simulink model "x00_AeroDynamicModelMainAssembly"  (R2016a)
settings: Solver=ode23t  StartTime=0.0  StopTime=10.0  MaxStep=0.1  RelTol=1e-3
model workspace: external: MATLAB File C:\Users\szhang\2016 ACT- Quanser\Aero Dynamic Model Export\x00_AeroDynamicModelMainAssembly_DataFile1.m (data not in the file)
undefined symbols (not defined in the file or in its folder): _AICAD8418WBRMZ_Default_sldprt, _AICBCR421UW67_Default_sldprt, _C0402100n25V_Default_sldprt, _C040210n25V_Default_sldprt, _C040212p50VC0G_Default_sldprt, _C06031u35V_Default_sldprt, _C06032u216V_Default_sldprt, _C100U50VEEEFC1H101P_Default_sldprt, _C12064u750V_01_sldprt, _C121010U50V_Default_sldprt, _COMMCYUSB2014BZXC_Default_sldprt, _COMMON_01_sldprt, _COMMON_Default_sldprt, _CONNFUSBBSMT_01_sldprt, _CONNMDF3A12P2DSA_Default_sldprt, _CONNMDF3A4P2DSA_Default_sldprt, _CONNMDF3A6P2DS_Default_sldprt, _CONNMDF3A9P2DS_Default_sldprt, _CONNMODULAR8P8CTOP_Default_sldprt, _CONNPJ102BH_Default_sldprt, _CP6100U50VC0G_Default_sldprt, _CPLD5M80ZE64C5_Default_sldprt, _DB560C13F_01_sldprt, _Default_sldprt, _DSMBJ5361BTP_Default_sldprt, _EEPROMAT24CM01_Default_sldprt, _FBBLM21PG221SN1D_01_sldprt, _FBMPZ2012S601A_01_sldprt, _LED3mmRedGreenRA_Default_sldprt, _LEDLTRBGFSFRedGreenBlue_Default_sldprt, _LOGICNCP361SNT1G_Default_sldprt, _LOGICNOTSN74LVC3G14DCU_Default_sldprt, _OPL6206QTR_Default_sldprt, _OSC40000MHZ_Default_sldprt, _R0402100K_Default_sldprt, _R040210K0_Default_sldprt, _R04021K00_Default_sldprt, _R0402200R_Default_sldprt, _R040222R0_Default_sldprt, _R04026K04_Default_sldprt, _R0402DNP_Default_sldprt, _RA40R0_Default_sldprt, _RA41K005, _TP16258543_01_sldprt, _TVSUNI28V_Default_sldprt, _TVSUNI53V_Default_sldprt, _VREGAP733333SAG7_Default_sldprt, _VREGLTM8022EVPBF_Default_sldprt, _VREGPAM3112DAB120_Default_sldprt, _VREGTPS79318DBVR_01_sldprt, _XTAL192MHZNX2520SA_Default_sldprt, BGA121, CAP, CEEEFC1H101P, CONNFUSBBSMT, CONNMDF3A12P2DSA, CONNMDF3A4P2DSA, CONNMDF3A6P2DS, CONNMDF3A9P2DS, CONNModular8P8C ... (+31)
libraries: sm_lib x1879, nesl_utility x1
(part 29 of 35)

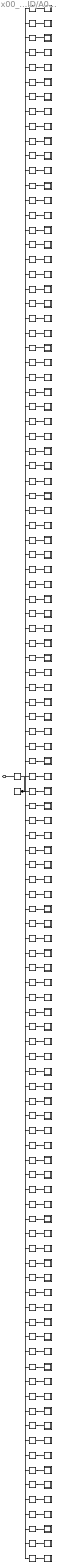
== system x00_AeroDynamicModelMainAssembly/x03_Aero_Dynamic_Model_Pivot_1_RIGID/A002_759_1_RIGID/A002_758_1_RIGID/C006_285_1_RIGID ==
  C006_285_1_RIGID : Subsystem
  CEEEFC1H101P_C100U50VEEEFC1H101P_1_RIGID : Subsystem
  CONNMDF3A6P2DS_CONNMDF3A6P2DS_1_RIGID : Subsystem
  CONNMDF3A6P2DS_CONNMDF3A6P2DS_2_RIGID : Subsystem
  CONNMDF3A9P2DS_CONNMDF3A9P2DS_1_RIGID : Subsystem
  DDO214AA_DSMBJ5361BTP_1_RIGID : Subsystem
  DDO214AB_DB560C13F_1_RIGID : Subsystem
  LGA16_3x3x086mm_ACCGYROLSM6DS0_1_RIGID : Subsystem
  MSOP10_COMMON_1_RIGID : Subsystem
  MSOP8Q_AICAD8418WBRMZ_1_RIGID : Subsystem
  MSOP8Q_AICAD8418WBRMZ_2_RIGID : Subsystem
  MSOP8Q_AICAD8418WBRMZ_3_RIGID : Subsystem
  MSOP8Q_AICAD8418WBRMZ_4_RIGID : Subsystem
  OSCECS20xx_OSC40000MHZ_1_RIGID : Subsystem
  RARRAYYC124_RA40R0_1_RIGID : Subsystem
  RARRAYYC124_RA40R0_2_RIGID : Subsystem
  RARRAYYC124_RA40R0_3_RIGID : Subsystem
  RARRAYYC124_RA40R0_4_RIGID : Subsystem
  RARRAYYC124_RA41K005_1_RIGID : Subsystem
  RARRAYYC124_RA41K005_2_RIGID : Subsystem
  ReferenceFrame : sm_lib/Frames and Transforms/Reference Frame
  SOT235_COMMON_1_RIGID : Subsystem
  SOT235_COMMON_2_RIGID : Subsystem
  SOT23_COMMON_1_RIGID : Subsystem
  SOT23_COMMON_2_RIGID : Subsystem
  SOT23_COMMON_3_RIGID : Subsystem
  TP16258543_TP16258543_1_RIGID : Subsystem
  TP16258543_TP16258543_2_RIGID : Subsystem
  TP16258543_TP16258543_3_RIGID : Subsystem
  TP16258543_TP16258543_4_RIGID : Subsystem
  TP16258543_TP16258543_5_RIGID : Subsystem
  TP16258543_TP16258543_6_RIGID : Subsystem
  TQFP144Max_V_CPLD_ground_pins_CPLD5M1270ZT144C5N_1_RIGID : Subsystem
  Transform : sm_lib/Frames and Transforms/Rigid Transform  TranslationMethod=Cartesian  TranslationLengthUnit=in  TranslationStandardAxis=+Z  TranslationStandardOffset=0  TranslationCartesianOffset=smiData.RigidTransform(427).translation  TranslationROffset=0  TranslationROffsetUnits=m  TranslationZOffset=0  TranslationZOffsetUnits=m  TranslationThetaOffset=0  TranslationThetaOffsetUnits=deg  RotationMethod=ArbitraryAxis  RotationAngleUnits=rad  RotationStandardAxis=+Z  RotationAngle=smiData.RigidTransform(427).angle  RotationArbitraryAxis=smiData.RigidTransform(427).axis  FollAlignAxisA=+X  BaseAlignAxisA=+Y  FollAlignAxisB=+Y  BaseAlignAxisB=+Z  RotationSequenceAxes=FollowerAxes  RotationSequence=XYX  RotationSequenceAngles=[0 0 0]  RotationSequenceAnglesUnits=deg  RotationMatrix=[1 0 0; 0 1 0; 0 0 1]
  Transform1 : sm_lib/Frames and Transforms/Rigid Transform  TranslationMethod=Cartesian  TranslationLengthUnit=in  TranslationStandardAxis=+Z  TranslationStandardOffset=0  TranslationCartesianOffset=smiData.RigidTransform(428).translation  TranslationROffset=0  TranslationROffsetUnits=m  TranslationZOffset=0  TranslationZOffsetUnits=m  TranslationThetaOffset=0  TranslationThetaOffsetUnits=deg  RotationMethod=ArbitraryAxis  RotationAngleUnits=rad  RotationStandardAxis=+Z  RotationAngle=smiData.RigidTransform(428).angle  RotationArbitraryAxis=smiData.RigidTransform(428).axis  FollAlignAxisA=+X  BaseAlignAxisA=+Y  FollAlignAxisB=+Y  BaseAlignAxisB=+Z  RotationSequenceAxes=FollowerAxes  RotationSequence=XYX  RotationSequenceAngles=[0 0 0]  RotationSequenceAnglesUnits=deg  RotationMatrix=[1 0 0; 0 1 0; 0 0 1]
  Transform10 : sm_lib/Frames and Transforms/Rigid Transform  TranslationMethod=Cartesian  TranslationLengthUnit=in  TranslationStandardAxis=+Z  TranslationStandardOffset=0  TranslationCartesianOffset=smiData.RigidTransform(437).translation  TranslationROffset=0  TranslationROffsetUnits=m  TranslationZOffset=0  TranslationZOffsetUnits=m  TranslationThetaOffset=0  TranslationThetaOffsetUnits=deg  RotationMethod=ArbitraryAxis  RotationAngleUnits=rad  RotationStandardAxis=+Z  RotationAngle=smiData.RigidTransform(437).angle  RotationArbitraryAxis=smiData.RigidTransform(437).axis  FollAlignAxisA=+X  BaseAlignAxisA=+Y  FollAlignAxisB=+Y  BaseAlignAxisB=+Z  RotationSequenceAxes=FollowerAxes  RotationSequence=XYX  RotationSequenceAngles=[0 0 0]  RotationSequenceAnglesUnits=deg  RotationMatrix=[1 0 0; 0 1 0; 0 0 1]
  Transform100 : sm_lib/Frames and Transforms/Rigid Transform  TranslationMethod=Cartesian  TranslationLengthUnit=in  TranslationStandardAxis=+Z  TranslationStandardOffset=0  TranslationCartesianOffset=smiData.RigidTransform(527).translation  TranslationROffset=0  TranslationROffsetUnits=m  TranslationZOffset=0  TranslationZOffsetUnits=m  TranslationThetaOffset=0  TranslationThetaOffsetUnits=deg  RotationMethod=ArbitraryAxis  RotationAngleUnits=rad  RotationStandardAxis=+Z  RotationAngle=smiData.RigidTransform(527).angle  RotationArbitraryAxis=smiData.RigidTransform(527).axis  FollAlignAxisA=+X  BaseAlignAxisA=+Y  FollAlignAxisB=+Y  BaseAlignAxisB=+Z  RotationSequenceAxes=FollowerAxes  RotationSequence=XYX  RotationSequenceAngles=[0 0 0]  RotationSequenceAnglesUnits=deg  RotationMatrix=[1 0 0; 0 1 0; 0 0 1]
  Transform101 : sm_lib/Frames and Transforms/Rigid Transform  TranslationMethod=Cartesian  TranslationLengthUnit=in  TranslationStandardAxis=+Z  TranslationStandardOffset=0  TranslationCartesianOffset=smiData.RigidTransform(528).translation  TranslationROffset=0  TranslationROffsetUnits=m  TranslationZOffset=0  TranslationZOffsetUnits=m  TranslationThetaOffset=0  TranslationThetaOffsetUnits=deg  RotationMethod=ArbitraryAxis  RotationAngleUnits=rad  RotationStandardAxis=+Z  RotationAngle=smiData.RigidTransform(528).angle  RotationArbitraryAxis=smiData.RigidTransform(528).axis  FollAlignAxisA=+X  BaseAlignAxisA=+Y  FollAlignAxisB=+Y  BaseAlignAxisB=+Z  RotationSequenceAxes=FollowerAxes  RotationSequence=XYX  RotationSequenceAngles=[0 0 0]  RotationSequenceAnglesUnits=deg  RotationMatrix=[1 0 0; 0 1 0; 0 0 1]
  Transform102 : sm_lib/Frames and Transforms/Rigid Transform  TranslationMethod=Cartesian  TranslationLengthUnit=in  TranslationStandardAxis=+Z  TranslationStandardOffset=0  TranslationCartesianOffset=smiData.RigidTransform(529).translation  TranslationROffset=0  TranslationROffsetUnits=m  TranslationZOffset=0  TranslationZOffsetUnits=m  TranslationThetaOffset=0  TranslationThetaOffsetUnits=deg  RotationMethod=ArbitraryAxis  RotationAngleUnits=rad  RotationStandardAxis=+Z  RotationAngle=smiData.RigidTransform(529).angle  RotationArbitraryAxis=smiData.RigidTransform(529).axis  FollAlignAxisA=+X  BaseAlignAxisA=+Y  FollAlignAxisB=+Y  BaseAlignAxisB=+Z  RotationSequenceAxes=FollowerAxes  RotationSequence=XYX  RotationSequenceAngles=[0 0 0]  RotationSequenceAnglesUnits=deg  RotationMatrix=[1 0 0; 0 1 0; 0 0 1]
  Transform103 : sm_lib/Frames and Transforms/Rigid Transform  TranslationMethod=Cartesian  TranslationLengthUnit=in  TranslationStandardAxis=+Z  TranslationStandardOffset=0  TranslationCartesianOffset=smiData.RigidTransform(530).translation  TranslationROffset=0  TranslationROffsetUnits=m  TranslationZOffset=0  TranslationZOffsetUnits=m  TranslationThetaOffset=0  TranslationThetaOffsetUnits=deg  RotationMethod=ArbitraryAxis  RotationAngleUnits=rad  RotationStandardAxis=+Z  RotationAngle=smiData.RigidTransform(530).angle  RotationArbitraryAxis=smiData.RigidTransform(530).axis  FollAlignAxisA=+X  BaseAlignAxisA=+Y  FollAlignAxisB=+Y  BaseAlignAxisB=+Z  RotationSequenceAxes=FollowerAxes  RotationSequence=XYX  RotationSequenceAngles=[0 0 0]  RotationSequenceAnglesUnits=deg  RotationMatrix=[1 0 0; 0 1 0; 0 0 1]
  Transform104 : sm_lib/Frames and Transforms/Rigid Transform  TranslationMethod=Cartesian  TranslationLengthUnit=in  TranslationStandardAxis=+Z  TranslationStandardOffset=0  TranslationCartesianOffset=smiData.RigidTransform(531).translation  TranslationROffset=0  TranslationROffsetUnits=m  TranslationZOffset=0  TranslationZOffsetUnits=m  TranslationThetaOffset=0  TranslationThetaOffsetUnits=deg  RotationMethod=ArbitraryAxis  RotationAngleUnits=rad  RotationStandardAxis=+Z  RotationAngle=smiData.RigidTransform(531).angle  RotationArbitraryAxis=smiData.RigidTransform(531).axis  FollAlignAxisA=+X  BaseAlignAxisA=+Y  FollAlignAxisB=+Y  BaseAlignAxisB=+Z  RotationSequenceAxes=FollowerAxes  RotationSequence=XYX  RotationSequenceAngles=[0 0 0]  RotationSequenceAnglesUnits=deg  RotationMatrix=[1 0 0; 0 1 0; 0 0 1]
  Transform105 : sm_lib/Frames and Transforms/Rigid Transform  TranslationMethod=Cartesian  TranslationLengthUnit=in  TranslationStandardAxis=+Z  TranslationStandardOffset=0  TranslationCartesianOffset=smiData.RigidTransform(532).translation  TranslationROffset=0  TranslationROffsetUnits=m  TranslationZOffset=0  TranslationZOffsetUnits=m  TranslationThetaOffset=0  TranslationThetaOffsetUnits=deg  RotationMethod=ArbitraryAxis  RotationAngleUnits=rad  RotationStandardAxis=+Z  RotationAngle=smiData.RigidTransform(532).angle  RotationArbitraryAxis=smiData.RigidTransform(532).axis  FollAlignAxisA=+X  BaseAlignAxisA=+Y  FollAlignAxisB=+Y  BaseAlignAxisB=+Z  RotationSequenceAxes=FollowerAxes  RotationSequence=XYX  RotationSequenceAngles=[0 0 0]  RotationSequenceAnglesUnits=deg  RotationMatrix=[1 0 0; 0 1 0; 0 0 1]
  Transform106 : sm_lib/Frames and Transforms/Rigid Transform  TranslationMethod=Cartesian  TranslationLengthUnit=in  TranslationStandardAxis=+Z  TranslationStandardOffset=0  TranslationCartesianOffset=smiData.RigidTransform(533).translation  TranslationROffset=0  TranslationROffsetUnits=m  TranslationZOffset=0  TranslationZOffsetUnits=m  TranslationThetaOffset=0  TranslationThetaOffsetUnits=deg  RotationMethod=ArbitraryAxis  RotationAngleUnits=rad  RotationStandardAxis=+Z  RotationAngle=smiData.RigidTransform(533).angle  RotationArbitraryAxis=smiData.RigidTransform(533).axis  FollAlignAxisA=+X  BaseAlignAxisA=+Y  FollAlignAxisB=+Y  BaseAlignAxisB=+Z  RotationSequenceAxes=FollowerAxes  RotationSequence=XYX  RotationSequenceAngles=[0 0 0]  RotationSequenceAnglesUnits=deg  RotationMatrix=[1 0 0; 0 1 0; 0 0 1]
  Transform11 : sm_lib/Frames and Transforms/Rigid Transform  TranslationMethod=Cartesian  TranslationLengthUnit=in  TranslationStandardAxis=+Z  TranslationStandardOffset=0  TranslationCartesianOffset=smiData.RigidTransform(438).translation  TranslationROffset=0  TranslationROffsetUnits=m  TranslationZOffset=0  TranslationZOffsetUnits=m  TranslationThetaOffset=0  TranslationThetaOffsetUnits=deg  RotationMethod=ArbitraryAxis  RotationAngleUnits=rad  RotationStandardAxis=+Z  RotationAngle=smiData.RigidTransform(438).angle  RotationArbitraryAxis=smiData.RigidTransform(438).axis  FollAlignAxisA=+X  BaseAlignAxisA=+Y  FollAlignAxisB=+Y  BaseAlignAxisB=+Z  RotationSequenceAxes=FollowerAxes  RotationSequence=XYX  RotationSequenceAngles=[0 0 0]  RotationSequenceAnglesUnits=deg  RotationMatrix=[1 0 0; 0 1 0; 0 0 1]
  Transform12 : sm_lib/Frames and Transforms/Rigid Transform  TranslationMethod=Cartesian  TranslationLengthUnit=in  TranslationStandardAxis=+Z  TranslationStandardOffset=0  TranslationCartesianOffset=smiData.RigidTransform(439).translation  TranslationROffset=0  TranslationROffsetUnits=m  TranslationZOffset=0  TranslationZOffsetUnits=m  TranslationThetaOffset=0  TranslationThetaOffsetUnits=deg  RotationMethod=ArbitraryAxis  RotationAngleUnits=rad  RotationStandardAxis=+Z  RotationAngle=smiData.RigidTransform(439).angle  RotationArbitraryAxis=smiData.RigidTransform(439).axis  FollAlignAxisA=+X  BaseAlignAxisA=+Y  FollAlignAxisB=+Y  BaseAlignAxisB=+Z  RotationSequenceAxes=FollowerAxes  RotationSequence=XYX  RotationSequenceAngles=[0 0 0]  RotationSequenceAnglesUnits=deg  RotationMatrix=[1 0 0; 0 1 0; 0 0 1]
  Transform13 : sm_lib/Frames and Transforms/Rigid Transform  TranslationMethod=Cartesian  TranslationLengthUnit=in  TranslationStandardAxis=+Z  TranslationStandardOffset=0  TranslationCartesianOffset=smiData.RigidTransform(440).translation  TranslationROffset=0  TranslationROffsetUnits=m  TranslationZOffset=0  TranslationZOffsetUnits=m  TranslationThetaOffset=0  TranslationThetaOffsetUnits=deg  RotationMethod=ArbitraryAxis  RotationAngleUnits=rad  RotationStandardAxis=+Z  RotationAngle=smiData.RigidTransform(440).angle  RotationArbitraryAxis=smiData.RigidTransform(440).axis  FollAlignAxisA=+X  BaseAlignAxisA=+Y  FollAlignAxisB=+Y  BaseAlignAxisB=+Z  RotationSequenceAxes=FollowerAxes  RotationSequence=XYX  RotationSequenceAngles=[0 0 0]  RotationSequenceAnglesUnits=deg  RotationMatrix=[1 0 0; 0 1 0; 0 0 1]
  Transform14 : sm_lib/Frames and Transforms/Rigid Transform  TranslationMethod=Cartesian  TranslationLengthUnit=in  TranslationStandardAxis=+Z  TranslationStandardOffset=0  TranslationCartesianOffset=smiData.RigidTransform(441).translation  TranslationROffset=0  TranslationROffsetUnits=m  TranslationZOffset=0  TranslationZOffsetUnits=m  TranslationThetaOffset=0  TranslationThetaOffsetUnits=deg  RotationMethod=ArbitraryAxis  RotationAngleUnits=rad  RotationStandardAxis=+Z  RotationAngle=smiData.RigidTransform(441).angle  RotationArbitraryAxis=smiData.RigidTransform(441).axis  FollAlignAxisA=+X  BaseAlignAxisA=+Y  FollAlignAxisB=+Y  BaseAlignAxisB=+Z  RotationSequenceAxes=FollowerAxes  RotationSequence=XYX  RotationSequenceAngles=[0 0 0]  RotationSequenceAnglesUnits=deg  RotationMatrix=[1 0 0; 0 1 0; 0 0 1]
  Transform15 : sm_lib/Frames and Transforms/Rigid Transform  TranslationMethod=Cartesian  TranslationLengthUnit=in  TranslationStandardAxis=+Z  TranslationStandardOffset=0  TranslationCartesianOffset=smiData.RigidTransform(442).translation  TranslationROffset=0  TranslationROffsetUnits=m  TranslationZOffset=0  TranslationZOffsetUnits=m  TranslationThetaOffset=0  TranslationThetaOffsetUnits=deg  RotationMethod=ArbitraryAxis  RotationAngleUnits=rad  RotationStandardAxis=+Z  RotationAngle=smiData.RigidTransform(442).angle  RotationArbitraryAxis=smiData.RigidTransform(442).axis  FollAlignAxisA=+X  BaseAlignAxisA=+Y  FollAlignAxisB=+Y  BaseAlignAxisB=+Z  RotationSequenceAxes=FollowerAxes  RotationSequence=XYX  RotationSequenceAngles=[0 0 0]  RotationSequenceAnglesUnits=deg  RotationMatrix=[1 0 0; 0 1 0; 0 0 1]
  Transform16 : sm_lib/Frames and Transforms/Rigid Transform  TranslationMethod=Cartesian  TranslationLengthUnit=in  TranslationStandardAxis=+Z  TranslationStandardOffset=0  TranslationCartesianOffset=smiData.RigidTransform(443).translation  TranslationROffset=0  TranslationROffsetUnits=m  TranslationZOffset=0  TranslationZOffsetUnits=m  TranslationThetaOffset=0  TranslationThetaOffsetUnits=deg  RotationMethod=ArbitraryAxis  RotationAngleUnits=rad  RotationStandardAxis=+Z  RotationAngle=smiData.RigidTransform(443).angle  RotationArbitraryAxis=smiData.RigidTransform(443).axis  FollAlignAxisA=+X  BaseAlignAxisA=+Y  FollAlignAxisB=+Y  BaseAlignAxisB=+Z  RotationSequenceAxes=FollowerAxes  RotationSequence=XYX  RotationSequenceAngles=[0 0 0]  RotationSequenceAnglesUnits=deg  RotationMatrix=[1 0 0; 0 1 0; 0 0 1]
  Transform17 : sm_lib/Frames and Transforms/Rigid Transform  TranslationMethod=Cartesian  TranslationLengthUnit=in  TranslationStandardAxis=+Z  TranslationStandardOffset=0  TranslationCartesianOffset=smiData.RigidTransform(444).translation  TranslationROffset=0  TranslationROffsetUnits=m  TranslationZOffset=0  TranslationZOffsetUnits=m  TranslationThetaOffset=0  TranslationThetaOffsetUnits=deg  RotationMethod=ArbitraryAxis  RotationAngleUnits=rad  RotationStandardAxis=+Z  RotationAngle=smiData.RigidTransform(444).angle  RotationArbitraryAxis=smiData.RigidTransform(444).axis  FollAlignAxisA=+X  BaseAlignAxisA=+Y  FollAlignAxisB=+Y  BaseAlignAxisB=+Z  RotationSequenceAxes=FollowerAxes  RotationSequence=XYX  RotationSequenceAngles=[0 0 0]  RotationSequenceAnglesUnits=deg  RotationMatrix=[1 0 0; 0 1 0; 0 0 1]
  Transform18 : sm_lib/Frames and Transforms/Rigid Transform  TranslationMethod=Cartesian  TranslationLengthUnit=in  TranslationStandardAxis=+Z  TranslationStandardOffset=0  TranslationCartesianOffset=smiData.RigidTransform(445).translation  TranslationROffset=0  TranslationROffsetUnits=m  TranslationZOffset=0  TranslationZOffsetUnits=m  TranslationThetaOffset=0  TranslationThetaOffsetUnits=deg  RotationMethod=ArbitraryAxis  RotationAngleUnits=rad  RotationStandardAxis=+Z  RotationAngle=smiData.RigidTransform(445).angle  RotationArbitraryAxis=smiData.RigidTransform(445).axis  FollAlignAxisA=+X  BaseAlignAxisA=+Y  FollAlignAxisB=+Y  BaseAlignAxisB=+Z  RotationSequenceAxes=FollowerAxes  RotationSequence=XYX  RotationSequenceAngles=[0 0 0]  RotationSequenceAnglesUnits=deg  RotationMatrix=[1 0 0; 0 1 0; 0 0 1]
  Transform19 : sm_lib/Frames and Transforms/Rigid Transform  TranslationMethod=Cartesian  TranslationLengthUnit=in  TranslationStandardAxis=+Z  TranslationStandardOffset=0  TranslationCartesianOffset=smiData.RigidTransform(446).translation  TranslationROffset=0  TranslationROffsetUnits=m  TranslationZOffset=0  TranslationZOffsetUnits=m  TranslationThetaOffset=0  TranslationThetaOffsetUnits=deg  RotationMethod=ArbitraryAxis  RotationAngleUnits=rad  RotationStandardAxis=+Z  RotationAngle=smiData.RigidTransform(446).angle  RotationArbitraryAxis=smiData.RigidTransform(446).axis  FollAlignAxisA=+X  BaseAlignAxisA=+Y  FollAlignAxisB=+Y  BaseAlignAxisB=+Z  RotationSequenceAxes=FollowerAxes  RotationSequence=XYX  RotationSequenceAngles=[0 0 0]  RotationSequenceAnglesUnits=deg  RotationMatrix=[1 0 0; 0 1 0; 0 0 1]
  Transform2 : sm_lib/Frames and Transforms/Rigid Transform  TranslationMethod=Cartesian  TranslationLengthUnit=in  TranslationStandardAxis=+Z  TranslationStandardOffset=0  TranslationCartesianOffset=smiData.RigidTransform(429).translation  TranslationROffset=0  TranslationROffsetUnits=m  TranslationZOffset=0  TranslationZOffsetUnits=m  TranslationThetaOffset=0  TranslationThetaOffsetUnits=deg  RotationMethod=ArbitraryAxis  RotationAngleUnits=rad  RotationStandardAxis=+Z  RotationAngle=smiData.RigidTransform(429).angle  RotationArbitraryAxis=smiData.RigidTransform(429).axis  FollAlignAxisA=+X  BaseAlignAxisA=+Y  FollAlignAxisB=+Y  BaseAlignAxisB=+Z  RotationSequenceAxes=FollowerAxes  RotationSequence=XYX  RotationSequenceAngles=[0 0 0]  RotationSequenceAnglesUnits=deg  RotationMatrix=[1 0 0; 0 1 0; 0 0 1]
  Transform20 : sm_lib/Frames and Transforms/Rigid Transform  TranslationMethod=Cartesian  TranslationLengthUnit=in  TranslationStandardAxis=+Z  TranslationStandardOffset=0  TranslationCartesianOffset=smiData.RigidTransform(447).translation  TranslationROffset=0  TranslationROffsetUnits=m  TranslationZOffset=0  TranslationZOffsetUnits=m  TranslationThetaOffset=0  TranslationThetaOffsetUnits=deg  RotationMethod=ArbitraryAxis  RotationAngleUnits=rad  RotationStandardAxis=+Z  RotationAngle=smiData.RigidTransform(447).angle  RotationArbitraryAxis=smiData.RigidTransform(447).axis  FollAlignAxisA=+X  BaseAlignAxisA=+Y  FollAlignAxisB=+Y  BaseAlignAxisB=+Z  RotationSequenceAxes=FollowerAxes  RotationSequence=XYX  RotationSequenceAngles=[0 0 0]  RotationSequenceAnglesUnits=deg  RotationMatrix=[1 0 0; 0 1 0; 0 0 1]
  Transform21 : sm_lib/Frames and Transforms/Rigid Transform  TranslationMethod=Cartesian  TranslationLengthUnit=in  TranslationStandardAxis=+Z  TranslationStandardOffset=0  TranslationCartesianOffset=smiData.RigidTransform(448).translation  TranslationROffset=0  TranslationROffsetUnits=m  TranslationZOffset=0  TranslationZOffsetUnits=m  TranslationThetaOffset=0  TranslationThetaOffsetUnits=deg  RotationMethod=ArbitraryAxis  RotationAngleUnits=rad  RotationStandardAxis=+Z  RotationAngle=smiData.RigidTransform(448).angle  RotationArbitraryAxis=smiData.RigidTransform(448).axis  FollAlignAxisA=+X  BaseAlignAxisA=+Y  FollAlignAxisB=+Y  BaseAlignAxisB=+Z  RotationSequenceAxes=FollowerAxes  RotationSequence=XYX  RotationSequenceAngles=[0 0 0]  RotationSequenceAnglesUnits=deg  RotationMatrix=[1 0 0; 0 1 0; 0 0 1]
  Transform22 : sm_lib/Frames and Transforms/Rigid Transform  TranslationMethod=Cartesian  TranslationLengthUnit=in  TranslationStandardAxis=+Z  TranslationStandardOffset=0  TranslationCartesianOffset=smiData.RigidTransform(449).translation  TranslationROffset=0  TranslationROffsetUnits=m  TranslationZOffset=0  TranslationZOffsetUnits=m  TranslationThetaOffset=0  TranslationThetaOffsetUnits=deg  RotationMethod=ArbitraryAxis  RotationAngleUnits=rad  RotationStandardAxis=+Z  RotationAngle=smiData.RigidTransform(449).angle  RotationArbitraryAxis=smiData.RigidTransform(449).axis  FollAlignAxisA=+X  BaseAlignAxisA=+Y  FollAlignAxisB=+Y  BaseAlignAxisB=+Z  RotationSequenceAxes=FollowerAxes  RotationSequence=XYX  RotationSequenceAngles=[0 0 0]  RotationSequenceAnglesUnits=deg  RotationMatrix=[1 0 0; 0 1 0; 0 0 1]
  Transform23 : sm_lib/Frames and Transforms/Rigid Transform  TranslationMethod=Cartesian  TranslationLengthUnit=in  TranslationStandardAxis=+Z  TranslationStandardOffset=0  TranslationCartesianOffset=smiData.RigidTransform(450).translation  TranslationROffset=0  TranslationROffsetUnits=m  TranslationZOffset=0  TranslationZOffsetUnits=m  TranslationThetaOffset=0  TranslationThetaOffsetUnits=deg  RotationMethod=ArbitraryAxis  RotationAngleUnits=rad  RotationStandardAxis=+Z  RotationAngle=smiData.RigidTransform(450).angle  RotationArbitraryAxis=smiData.RigidTransform(450).axis  FollAlignAxisA=+X  BaseAlignAxisA=+Y  FollAlignAxisB=+Y  BaseAlignAxisB=+Z  RotationSequenceAxes=FollowerAxes  RotationSequence=XYX  RotationSequenceAngles=[0 0 0]  RotationSequenceAnglesUnits=deg  RotationMatrix=[1 0 0; 0 1 0; 0 0 1]
  Transform24 : sm_lib/Frames and Transforms/Rigid Transform  TranslationMethod=Cartesian  TranslationLengthUnit=in  TranslationStandardAxis=+Z  TranslationStandardOffset=0  TranslationCartesianOffset=smiData.RigidTransform(451).translation  TranslationROffset=0  TranslationROffsetUnits=m  TranslationZOffset=0  TranslationZOffsetUnits=m  TranslationThetaOffset=0  TranslationThetaOffsetUnits=deg  RotationMethod=ArbitraryAxis  RotationAngleUnits=rad  RotationStandardAxis=+Z  RotationAngle=smiData.RigidTransform(451).angle  RotationArbitraryAxis=smiData.RigidTransform(451).axis  FollAlignAxisA=+X  BaseAlignAxisA=+Y  FollAlignAxisB=+Y  BaseAlignAxisB=+Z  RotationSequenceAxes=FollowerAxes  RotationSequence=XYX  RotationSequenceAngles=[0 0 0]  RotationSequenceAnglesUnits=deg  RotationMatrix=[1 0 0; 0 1 0; 0 0 1]
  Transform25 : sm_lib/Frames and Transforms/Rigid Transform  TranslationMethod=Cartesian  TranslationLengthUnit=in  TranslationStandardAxis=+Z  TranslationStandardOffset=0  TranslationCartesianOffset=smiData.RigidTransform(452).translation  TranslationROffset=0  TranslationROffsetUnits=m  TranslationZOffset=0  TranslationZOffsetUnits=m  TranslationThetaOffset=0  TranslationThetaOffsetUnits=deg  RotationMethod=ArbitraryAxis  RotationAngleUnits=rad  RotationStandardAxis=+Z  RotationAngle=smiData.RigidTransform(452).angle  RotationArbitraryAxis=smiData.RigidTransform(452).axis  FollAlignAxisA=+X  BaseAlignAxisA=+Y  FollAlignAxisB=+Y  BaseAlignAxisB=+Z  RotationSequenceAxes=FollowerAxes  RotationSequence=XYX  RotationSequenceAngles=[0 0 0]  RotationSequenceAnglesUnits=deg  RotationMatrix=[1 0 0; 0 1 0; 0 0 1]
  Transform26 : sm_lib/Frames and Transforms/Rigid Transform  TranslationMethod=Cartesian  TranslationLengthUnit=in  TranslationStandardAxis=+Z  TranslationStandardOffset=0  TranslationCartesianOffset=smiData.RigidTransform(453).translation  TranslationROffset=0  TranslationROffsetUnits=m  TranslationZOffset=0  TranslationZOffsetUnits=m  TranslationThetaOffset=0  TranslationThetaOffsetUnits=deg  RotationMethod=ArbitraryAxis  RotationAngleUnits=rad  RotationStandardAxis=+Z  RotationAngle=smiData.RigidTransform(453).angle  RotationArbitraryAxis=smiData.RigidTransform(453).axis  FollAlignAxisA=+X  BaseAlignAxisA=+Y  FollAlignAxisB=+Y  BaseAlignAxisB=+Z  RotationSequenceAxes=FollowerAxes  RotationSequence=XYX  RotationSequenceAngles=[0 0 0]  RotationSequenceAnglesUnits=deg  RotationMatrix=[1 0 0; 0 1 0; 0 0 1]
  Transform27 : sm_lib/Frames and Transforms/Rigid Transform  TranslationMethod=Cartesian  TranslationLengthUnit=in  TranslationStandardAxis=+Z  TranslationStandardOffset=0  TranslationCartesianOffset=smiData.RigidTransform(454).translation  TranslationROffset=0  TranslationROffsetUnits=m  TranslationZOffset=0  TranslationZOffsetUnits=m  TranslationThetaOffset=0  TranslationThetaOffsetUnits=deg  RotationMethod=ArbitraryAxis  RotationAngleUnits=rad  RotationStandardAxis=+Z  RotationAngle=smiData.RigidTransform(454).angle  RotationArbitraryAxis=smiData.RigidTransform(454).axis  FollAlignAxisA=+X  BaseAlignAxisA=+Y  FollAlignAxisB=+Y  BaseAlignAxisB=+Z  RotationSequenceAxes=FollowerAxes  RotationSequence=XYX  RotationSequenceAngles=[0 0 0]  RotationSequenceAnglesUnits=deg  RotationMatrix=[1 0 0; 0 1 0; 0 0 1]
  Transform28 : sm_lib/Frames and Transforms/Rigid Transform  TranslationMethod=Cartesian  TranslationLengthUnit=in  TranslationStandardAxis=+Z  TranslationStandardOffset=0  TranslationCartesianOffset=smiData.RigidTransform(455).translation  TranslationROffset=0  TranslationROffsetUnits=m  TranslationZOffset=0  TranslationZOffsetUnits=m  TranslationThetaOffset=0  TranslationThetaOffsetUnits=deg  RotationMethod=ArbitraryAxis  RotationAngleUnits=rad  RotationStandardAxis=+Z  RotationAngle=smiData.RigidTransform(455).angle  RotationArbitraryAxis=smiData.RigidTransform(455).axis  FollAlignAxisA=+X  BaseAlignAxisA=+Y  FollAlignAxisB=+Y  BaseAlignAxisB=+Z  RotationSequenceAxes=FollowerAxes  RotationSequence=XYX  RotationSequenceAngles=[0 0 0]  RotationSequenceAnglesUnits=deg  RotationMatrix=[1 0 0; 0 1 0; 0 0 1]
  Transform29 : sm_lib/Frames and Transforms/Rigid Transform  TranslationMethod=Cartesian  TranslationLengthUnit=in  TranslationStandardAxis=+Z  TranslationStandardOffset=0  TranslationCartesianOffset=smiData.RigidTransform(456).translation  TranslationROffset=0  TranslationROffsetUnits=m  TranslationZOffset=0  TranslationZOffsetUnits=m  TranslationThetaOffset=0  TranslationThetaOffsetUnits=deg  RotationMethod=ArbitraryAxis  RotationAngleUnits=rad  RotationStandardAxis=+Z  RotationAngle=smiData.RigidTransform(456).angle  RotationArbitraryAxis=smiData.RigidTransform(456).axis  FollAlignAxisA=+X  BaseAlignAxisA=+Y  FollAlignAxisB=+Y  BaseAlignAxisB=+Z  RotationSequenceAxes=FollowerAxes  RotationSequence=XYX  RotationSequenceAngles=[0 0 0]  RotationSequenceAnglesUnits=deg  RotationMatrix=[1 0 0; 0 1 0; 0 0 1]
  Transform3 : sm_lib/Frames and Transforms/Rigid Transform  TranslationMethod=Cartesian  TranslationLengthUnit=in  TranslationStandardAxis=+Z  TranslationStandardOffset=0  TranslationCartesianOffset=smiData.RigidTransform(430).translation  TranslationROffset=0  TranslationROffsetUnits=m  TranslationZOffset=0  TranslationZOffsetUnits=m  TranslationThetaOffset=0  TranslationThetaOffsetUnits=deg  RotationMethod=ArbitraryAxis  RotationAngleUnits=rad  RotationStandardAxis=+Z  RotationAngle=smiData.RigidTransform(430).angle  RotationArbitraryAxis=smiData.RigidTransform(430).axis  FollAlignAxisA=+X  BaseAlignAxisA=+Y  FollAlignAxisB=+Y  BaseAlignAxisB=+Z  RotationSequenceAxes=FollowerAxes  RotationSequence=XYX  RotationSequenceAngles=[0 0 0]  RotationSequenceAnglesUnits=deg  RotationMatrix=[1 0 0; 0 1 0; 0 0 1]
  Transform30 : sm_lib/Frames and Transforms/Rigid Transform  TranslationMethod=Cartesian  TranslationLengthUnit=in  TranslationStandardAxis=+Z  TranslationStandardOffset=0  TranslationCartesianOffset=smiData.RigidTransform(457).translation  TranslationROffset=0  TranslationROffsetUnits=m  TranslationZOffset=0  TranslationZOffsetUnits=m  TranslationThetaOffset=0  TranslationThetaOffsetUnits=deg  RotationMethod=ArbitraryAxis  RotationAngleUnits=rad  RotationStandardAxis=+Z  RotationAngle=smiData.RigidTransform(457).angle  RotationArbitraryAxis=smiData.RigidTransform(457).axis  FollAlignAxisA=+X  BaseAlignAxisA=+Y  FollAlignAxisB=+Y  BaseAlignAxisB=+Z  RotationSequenceAxes=FollowerAxes  RotationSequence=XYX  RotationSequenceAngles=[0 0 0]  RotationSequenceAnglesUnits=deg  RotationMatrix=[1 0 0; 0 1 0; 0 0 1]
  Transform31 : sm_lib/Frames and Transforms/Rigid Transform  TranslationMethod=Cartesian  TranslationLengthUnit=in  TranslationStandardAxis=+Z  TranslationStandardOffset=0  TranslationCartesianOffset=smiData.RigidTransform(458).translation  TranslationROffset=0  TranslationROffsetUnits=m  TranslationZOffset=0  TranslationZOffsetUnits=m  TranslationThetaOffset=0  TranslationThetaOffsetUnits=deg  RotationMethod=ArbitraryAxis  RotationAngleUnits=rad  RotationStandardAxis=+Z  RotationAngle=smiData.RigidTransform(458).angle  RotationArbitraryAxis=smiData.RigidTransform(458).axis  FollAlignAxisA=+X  BaseAlignAxisA=+Y  FollAlignAxisB=+Y  BaseAlignAxisB=+Z  RotationSequenceAxes=FollowerAxes  RotationSequence=XYX  RotationSequenceAngles=[0 0 0]  RotationSequenceAnglesUnits=deg  RotationMatrix=[1 0 0; 0 1 0; 0 0 1]
  Transform32 : sm_lib/Frames and Transforms/Rigid Transform  TranslationMethod=Cartesian  TranslationLengthUnit=in  TranslationStandardAxis=+Z  TranslationStandardOffset=0  TranslationCartesianOffset=smiData.RigidTransform(459).translation  TranslationROffset=0  TranslationROffsetUnits=m  TranslationZOffset=0  TranslationZOffsetUnits=m  TranslationThetaOffset=0  TranslationThetaOffsetUnits=deg  RotationMethod=ArbitraryAxis  RotationAngleUnits=rad  RotationStandardAxis=+Z  RotationAngle=smiData.RigidTransform(459).angle  RotationArbitraryAxis=smiData.RigidTransform(459).axis  FollAlignAxisA=+X  BaseAlignAxisA=+Y  FollAlignAxisB=+Y  BaseAlignAxisB=+Z  RotationSequenceAxes=FollowerAxes  RotationSequence=XYX  RotationSequenceAngles=[0 0 0]  RotationSequenceAnglesUnits=deg  RotationMatrix=[1 0 0; 0 1 0; 0 0 1]
  Transform33 : sm_lib/Frames and Transforms/Rigid Transform  TranslationMethod=Cartesian  TranslationLengthUnit=in  TranslationStandardAxis=+Z  TranslationStandardOffset=0  TranslationCartesianOffset=smiData.RigidTransform(460).translation  TranslationROffset=0  TranslationROffsetUnits=m  TranslationZOffset=0  TranslationZOffsetUnits=m  TranslationThetaOffset=0  TranslationThetaOffsetUnits=deg  RotationMethod=ArbitraryAxis  RotationAngleUnits=rad  RotationStandardAxis=+Z  RotationAngle=smiData.RigidTransform(460).angle  RotationArbitraryAxis=smiData.RigidTransform(460).axis  FollAlignAxisA=+X  BaseAlignAxisA=+Y  FollAlignAxisB=+Y  BaseAlignAxisB=+Z  RotationSequenceAxes=FollowerAxes  RotationSequence=XYX  RotationSequenceAngles=[0 0 0]  RotationSequenceAnglesUnits=deg  RotationMatrix=[1 0 0; 0 1 0; 0 0 1]
  Transform34 : sm_lib/Frames and Transforms/Rigid Transform  TranslationMethod=Cartesian  TranslationLengthUnit=in  TranslationStandardAxis=+Z  TranslationStandardOffset=0  TranslationCartesianOffset=smiData.RigidTransform(461).translation  TranslationROffset=0  TranslationROffsetUnits=m  TranslationZOffset=0  TranslationZOffsetUnits=m  TranslationThetaOffset=0  TranslationThetaOffsetUnits=deg  RotationMethod=ArbitraryAxis  RotationAngleUnits=rad  RotationStandardAxis=+Z  RotationAngle=smiData.RigidTransform(461).angle  RotationArbitraryAxis=smiData.RigidTransform(461).axis  FollAlignAxisA=+X  BaseAlignAxisA=+Y  FollAlignAxisB=+Y  BaseAlignAxisB=+Z  RotationSequenceAxes=FollowerAxes  RotationSequence=XYX  RotationSequenceAngles=[0 0 0]  RotationSequenceAnglesUnits=deg  RotationMatrix=[1 0 0; 0 1 0; 0 0 1]
  Transform35 : sm_lib/Frames and Transforms/Rigid Transform  TranslationMethod=Cartesian  TranslationLengthUnit=in  TranslationStandardAxis=+Z  TranslationStandardOffset=0  TranslationCartesianOffset=smiData.RigidTransform(462).translation  TranslationROffset=0  TranslationROffsetUnits=m  TranslationZOffset=0  TranslationZOffsetUnits=m  TranslationThetaOffset=0  TranslationThetaOffsetUnits=deg  RotationMethod=ArbitraryAxis  RotationAngleUnits=rad  RotationStandardAxis=+Z  RotationAngle=smiData.RigidTransform(462).angle  RotationArbitraryAxis=smiData.RigidTransform(462).axis  FollAlignAxisA=+X  BaseAlignAxisA=+Y  FollAlignAxisB=+Y  BaseAlignAxisB=+Z  RotationSequenceAxes=FollowerAxes  RotationSequence=XYX  RotationSequenceAngles=[0 0 0]  RotationSequenceAnglesUnits=deg  RotationMatrix=[1 0 0; 0 1 0; 0 0 1]
  Transform36 : sm_lib/Frames and Transforms/Rigid Transform  TranslationMethod=Cartesian  TranslationLengthUnit=in  TranslationStandardAxis=+Z  TranslationStandardOffset=0  TranslationCartesianOffset=smiData.RigidTransform(463).translation  TranslationROffset=0  TranslationROffsetUnits=m  TranslationZOffset=0  TranslationZOffsetUnits=m  TranslationThetaOffset=0  TranslationThetaOffsetUnits=deg  RotationMethod=ArbitraryAxis  RotationAngleUnits=rad  RotationStandardAxis=+Z  RotationAngle=smiData.RigidTransform(463).angle  RotationArbitraryAxis=smiData.RigidTransform(463).axis  FollAlignAxisA=+X  BaseAlignAxisA=+Y  FollAlignAxisB=+Y  BaseAlignAxisB=+Z  RotationSequenceAxes=FollowerAxes  RotationSequence=XYX  RotationSequenceAngles=[0 0 0]  RotationSequenceAnglesUnits=deg  RotationMatrix=[1 0 0; 0 1 0; 0 0 1]
  Transform37 : sm_lib/Frames and Transforms/Rigid Transform  TranslationMethod=Cartesian  TranslationLengthUnit=in  TranslationStandardAxis=+Z  TranslationStandardOffset=0  TranslationCartesianOffset=smiData.RigidTransform(464).translation  TranslationROffset=0  TranslationROffsetUnits=m  TranslationZOffset=0  TranslationZOffsetUnits=m  TranslationThetaOffset=0  TranslationThetaOffsetUnits=deg  RotationMethod=ArbitraryAxis  RotationAngleUnits=rad  RotationStandardAxis=+Z  RotationAngle=smiData.RigidTransform(464).angle  RotationArbitraryAxis=smiData.RigidTransform(464).axis  FollAlignAxisA=+X  BaseAlignAxisA=+Y  FollAlignAxisB=+Y  BaseAlignAxisB=+Z  RotationSequenceAxes=FollowerAxes  RotationSequence=XYX  RotationSequenceAngles=[0 0 0]  RotationSequenceAnglesUnits=deg  RotationMatrix=[1 0 0; 0 1 0; 0 0 1]
  Transform38 : sm_lib/Frames and Transforms/Rigid Transform  TranslationMethod=Cartesian  TranslationLengthUnit=in  TranslationStandardAxis=+Z  TranslationStandardOffset=0  TranslationCartesianOffset=smiData.RigidTransform(465).translation  TranslationROffset=0  TranslationROffsetUnits=m  TranslationZOffset=0  TranslationZOffsetUnits=m  TranslationThetaOffset=0  TranslationThetaOffsetUnits=deg  RotationMethod=ArbitraryAxis  RotationAngleUnits=rad  RotationStandardAxis=+Z  RotationAngle=smiData.RigidTransform(465).angle  RotationArbitraryAxis=smiData.RigidTransform(465).axis  FollAlignAxisA=+X  BaseAlignAxisA=+Y  FollAlignAxisB=+Y  BaseAlignAxisB=+Z  RotationSequenceAxes=FollowerAxes  RotationSequence=XYX  RotationSequenceAngles=[0 0 0]  RotationSequenceAnglesUnits=deg  RotationMatrix=[1 0 0; 0 1 0; 0 0 1]
  Transform39 : sm_lib/Frames and Transforms/Rigid Transform  TranslationMethod=Cartesian  TranslationLengthUnit=in  TranslationStandardAxis=+Z  TranslationStandardOffset=0  TranslationCartesianOffset=smiData.RigidTransform(466).translation  TranslationROffset=0  TranslationROffsetUnits=m  TranslationZOffset=0  TranslationZOffsetUnits=m  TranslationThetaOffset=0  TranslationThetaOffsetUnits=deg  RotationMethod=ArbitraryAxis  RotationAngleUnits=rad  RotationStandardAxis=+Z  RotationAngle=smiData.RigidTransform(466).angle  RotationArbitraryAxis=smiData.RigidTransform(466).axis  FollAlignAxisA=+X  BaseAlignAxisA=+Y  FollAlignAxisB=+Y  BaseAlignAxisB=+Z  RotationSequenceAxes=FollowerAxes  RotationSequence=XYX  RotationSequenceAngles=[0 0 0]  RotationSequenceAnglesUnits=deg  RotationMatrix=[1 0 0; 0 1 0; 0 0 1]
  Transform4 : sm_lib/Frames and Transforms/Rigid Transform  TranslationMethod=Cartesian  TranslationLengthUnit=in  TranslationStandardAxis=+Z  TranslationStandardOffset=0  TranslationCartesianOffset=smiData.RigidTransform(431).translation  TranslationROffset=0  TranslationROffsetUnits=m  TranslationZOffset=0  TranslationZOffsetUnits=m  TranslationThetaOffset=0  TranslationThetaOffsetUnits=deg  RotationMethod=ArbitraryAxis  RotationAngleUnits=rad  RotationStandardAxis=+Z  RotationAngle=smiData.RigidTransform(431).angle  RotationArbitraryAxis=smiData.RigidTransform(431).axis  FollAlignAxisA=+X  BaseAlignAxisA=+Y  FollAlignAxisB=+Y  BaseAlignAxisB=+Z  RotationSequenceAxes=FollowerAxes  RotationSequence=XYX  RotationSequenceAngles=[0 0 0]  RotationSequenceAnglesUnits=deg  RotationMatrix=[1 0 0; 0 1 0; 0 0 1]
  Transform40 : sm_lib/Frames and Transforms/Rigid Transform  TranslationMethod=Cartesian  TranslationLengthUnit=in  TranslationStandardAxis=+Z  TranslationStandardOffset=0  TranslationCartesianOffset=smiData.RigidTransform(467).translation  TranslationROffset=0  TranslationROffsetUnits=m  TranslationZOffset=0  TranslationZOffsetUnits=m  TranslationThetaOffset=0  TranslationThetaOffsetUnits=deg  RotationMethod=ArbitraryAxis  RotationAngleUnits=rad  RotationStandardAxis=+Z  RotationAngle=smiData.RigidTransform(467).angle  RotationArbitraryAxis=smiData.RigidTransform(467).axis  FollAlignAxisA=+X  BaseAlignAxisA=+Y  FollAlignAxisB=+Y  BaseAlignAxisB=+Z  RotationSequenceAxes=FollowerAxes  RotationSequence=XYX  RotationSequenceAngles=[0 0 0]  RotationSequenceAnglesUnits=deg  RotationMatrix=[1 0 0; 0 1 0; 0 0 1]
  Transform41 : sm_lib/Frames and Transforms/Rigid Transform  TranslationMethod=Cartesian  TranslationLengthUnit=in  TranslationStandardAxis=+Z  TranslationStandardOffset=0  TranslationCartesianOffset=smiData.RigidTransform(468).translation  TranslationROffset=0  TranslationROffsetUnits=m  TranslationZOffset=0  TranslationZOffsetUnits=m  TranslationThetaOffset=0  TranslationThetaOffsetUnits=deg  RotationMethod=ArbitraryAxis  RotationAngleUnits=rad  RotationStandardAxis=+Z  RotationAngle=smiData.RigidTransform(468).angle  RotationArbitraryAxis=smiData.RigidTransform(468).axis  FollAlignAxisA=+X  BaseAlignAxisA=+Y  FollAlignAxisB=+Y  BaseAlignAxisB=+Z  RotationSequenceAxes=FollowerAxes  RotationSequence=XYX  RotationSequenceAngles=[0 0 0]  RotationSequenceAnglesUnits=deg  RotationMatrix=[1 0 0; 0 1 0; 0 0 1]
  Transform42 : sm_lib/Frames and Transforms/Rigid Transform  TranslationMethod=Cartesian  TranslationLengthUnit=in  TranslationStandardAxis=+Z  TranslationStandardOffset=0  TranslationCartesianOffset=smiData.RigidTransform(469).translation  TranslationROffset=0  TranslationROffsetUnits=m  TranslationZOffset=0  TranslationZOffsetUnits=m  TranslationThetaOffset=0  TranslationThetaOffsetUnits=deg  RotationMethod=ArbitraryAxis  RotationAngleUnits=rad  RotationStandardAxis=+Z  RotationAngle=smiData.RigidTransform(469).angle  RotationArbitraryAxis=smiData.RigidTransform(469).axis  FollAlignAxisA=+X  BaseAlignAxisA=+Y  FollAlignAxisB=+Y  BaseAlignAxisB=+Z  RotationSequenceAxes=FollowerAxes  RotationSequence=XYX  RotationSequenceAngles=[0 0 0]  RotationSequenceAnglesUnits=deg  RotationMatrix=[1 0 0; 0 1 0; 0 0 1]
  Transform43 : sm_lib/Frames and Transforms/Rigid Transform  TranslationMethod=Cartesian  TranslationLengthUnit=in  TranslationStandardAxis=+Z  TranslationStandardOffset=0  TranslationCartesianOffset=smiData.RigidTransform(470).translation  TranslationROffset=0  TranslationROffsetUnits=m  TranslationZOffset=0  TranslationZOffsetUnits=m  TranslationThetaOffset=0  TranslationThetaOffsetUnits=deg  RotationMethod=ArbitraryAxis  RotationAngleUnits=rad  RotationStandardAxis=+Z  RotationAngle=smiData.RigidTransform(470).angle  RotationArbitraryAxis=smiData.RigidTransform(470).axis  FollAlignAxisA=+X  BaseAlignAxisA=+Y  FollAlignAxisB=+Y  BaseAlignAxisB=+Z  RotationSequenceAxes=FollowerAxes  RotationSequence=XYX  RotationSequenceAngles=[0 0 0]  RotationSequenceAnglesUnits=deg  RotationMatrix=[1 0 0; 0 1 0; 0 0 1]
  Transform44 : sm_lib/Frames and Transforms/Rigid Transform  TranslationMethod=Cartesian  TranslationLengthUnit=in  TranslationStandardAxis=+Z  TranslationStandardOffset=0  TranslationCartesianOffset=smiData.RigidTransform(471).translation  TranslationROffset=0  TranslationROffsetUnits=m  TranslationZOffset=0  TranslationZOffsetUnits=m  TranslationThetaOffset=0  TranslationThetaOffsetUnits=deg  RotationMethod=ArbitraryAxis  RotationAngleUnits=rad  RotationStandardAxis=+Z  RotationAngle=smiData.RigidTransform(471).angle  RotationArbitraryAxis=smiData.RigidTransform(471).axis  FollAlignAxisA=+X  BaseAlignAxisA=+Y  FollAlignAxisB=+Y  BaseAlignAxisB=+Z  RotationSequenceAxes=FollowerAxes  RotationSequence=XYX  RotationSequenceAngles=[0 0 0]  RotationSequenceAnglesUnits=deg  RotationMatrix=[1 0 0; 0 1 0; 0 0 1]
  Transform45 : sm_lib/Frames and Transforms/Rigid Transform  TranslationMethod=Cartesian  TranslationLengthUnit=in  TranslationStandardAxis=+Z  TranslationStandardOffset=0  TranslationCartesianOffset=smiData.RigidTransform(472).translation  TranslationROffset=0  TranslationROffsetUnits=m  TranslationZOffset=0  TranslationZOffsetUnits=m  TranslationThetaOffset=0  TranslationThetaOffsetUnits=deg  RotationMethod=ArbitraryAxis  RotationAngleUnits=rad  RotationStandardAxis=+Z  RotationAngle=smiData.RigidTransform(472).angle  RotationArbitraryAxis=smiData.RigidTransform(472).axis  FollAlignAxisA=+X  BaseAlignAxisA=+Y  FollAlignAxisB=+Y  BaseAlignAxisB=+Z  RotationSequenceAxes=FollowerAxes  RotationSequence=XYX  RotationSequenceAngles=[0 0 0]  RotationSequenceAnglesUnits=deg  RotationMatrix=[1 0 0; 0 1 0; 0 0 1]
  Transform46 : sm_lib/Frames and Transforms/Rigid Transform  TranslationMethod=Cartesian  TranslationLengthUnit=in  TranslationStandardAxis=+Z  TranslationStandardOffset=0  TranslationCartesianOffset=smiData.RigidTransform(473).translation  TranslationROffset=0  TranslationROffsetUnits=m  TranslationZOffset=0  TranslationZOffsetUnits=m  TranslationThetaOffset=0  TranslationThetaOffsetUnits=deg  RotationMethod=ArbitraryAxis  RotationAngleUnits=rad  RotationStandardAxis=+Z  RotationAngle=smiData.RigidTransform(473).angle  RotationArbitraryAxis=smiData.RigidTransform(473).axis  FollAlignAxisA=+X  BaseAlignAxisA=+Y  FollAlignAxisB=+Y  BaseAlignAxisB=+Z  RotationSequenceAxes=FollowerAxes  RotationSequence=XYX  RotationSequenceAngles=[0 0 0]  RotationSequenceAnglesUnits=deg  RotationMatrix=[1 0 0; 0 1 0; 0 0 1]
  Transform47 : sm_lib/Frames and Transforms/Rigid Transform  TranslationMethod=Cartesian  TranslationLengthUnit=in  TranslationStandardAxis=+Z  TranslationStandardOffset=0  TranslationCartesianOffset=smiData.RigidTransform(474).translation  TranslationROffset=0  TranslationROffsetUnits=m  TranslationZOffset=0  TranslationZOffsetUnits=m  TranslationThetaOffset=0  TranslationThetaOffsetUnits=deg  RotationMethod=ArbitraryAxis  RotationAngleUnits=rad  RotationStandardAxis=+Z  RotationAngle=smiData.RigidTransform(474).angle  RotationArbitraryAxis=smiData.RigidTransform(474).axis  FollAlignAxisA=+X  BaseAlignAxisA=+Y  FollAlignAxisB=+Y  BaseAlignAxisB=+Z  RotationSequenceAxes=FollowerAxes  RotationSequence=XYX  RotationSequenceAngles=[0 0 0]  RotationSequenceAnglesUnits=deg  RotationMatrix=[1 0 0; 0 1 0; 0 0 1]
  Transform48 : sm_lib/Frames and Transforms/Rigid Transform  TranslationMethod=Cartesian  TranslationLengthUnit=in  TranslationStandardAxis=+Z  TranslationStandardOffset=0  TranslationCartesianOffset=smiData.RigidTransform(475).translation  TranslationROffset=0  TranslationROffsetUnits=m  TranslationZOffset=0  TranslationZOffsetUnits=m  TranslationThetaOffset=0  TranslationThetaOffsetUnits=deg  RotationMethod=ArbitraryAxis  RotationAngleUnits=rad  RotationStandardAxis=+Z  RotationAngle=smiData.RigidTransform(475).angle  RotationArbitraryAxis=smiData.RigidTransform(475).axis  FollAlignAxisA=+X  BaseAlignAxisA=+Y  FollAlignAxisB=+Y  BaseAlignAxisB=+Z  RotationSequenceAxes=FollowerAxes  RotationSequence=XYX  RotationSequenceAngles=[0 0 0]  RotationSequenceAnglesUnits=deg  RotationMatrix=[1 0 0; 0 1 0; 0 0 1]
  Transform49 : sm_lib/Frames and Transforms/Rigid Transform  TranslationMethod=Cartesian  TranslationLengthUnit=in  TranslationStandardAxis=+Z  TranslationStandardOffset=0  TranslationCartesianOffset=smiData.RigidTransform(476).translation  TranslationROffset=0  TranslationROffsetUnits=m  TranslationZOffset=0  TranslationZOffsetUnits=m  TranslationThetaOffset=0  TranslationThetaOffsetUnits=deg  RotationMethod=ArbitraryAxis  RotationAngleUnits=rad  RotationStandardAxis=+Z  RotationAngle=smiData.RigidTransform(476).angle  RotationArbitraryAxis=smiData.RigidTransform(476).axis  FollAlignAxisA=+X  BaseAlignAxisA=+Y  FollAlignAxisB=+Y  BaseAlignAxisB=+Z  RotationSequenceAxes=FollowerAxes  RotationSequence=XYX  RotationSequenceAngles=[0 0 0]  RotationSequenceAnglesUnits=deg  RotationMatrix=[1 0 0; 0 1 0; 0 0 1]
  Transform5 : sm_lib/Frames and Transforms/Rigid Transform  TranslationMethod=Cartesian  TranslationLengthUnit=in  TranslationStandardAxis=+Z  TranslationStandardOffset=0  TranslationCartesianOffset=smiData.RigidTransform(432).translation  TranslationROffset=0  TranslationROffsetUnits=m  TranslationZOffset=0  TranslationZOffsetUnits=m  TranslationThetaOffset=0  TranslationThetaOffsetUnits=deg  RotationMethod=ArbitraryAxis  RotationAngleUnits=rad  RotationStandardAxis=+Z  RotationAngle=smiData.RigidTransform(432).angle  RotationArbitraryAxis=smiData.RigidTransform(432).axis  FollAlignAxisA=+X  BaseAlignAxisA=+Y  FollAlignAxisB=+Y  BaseAlignAxisB=+Z  RotationSequenceAxes=FollowerAxes  RotationSequence=XYX  RotationSequenceAngles=[0 0 0]  RotationSequenceAnglesUnits=deg  RotationMatrix=[1 0 0; 0 1 0; 0 0 1]
  Transform50 : sm_lib/Frames and Transforms/Rigid Transform  TranslationMethod=Cartesian  TranslationLengthUnit=in  TranslationStandardAxis=+Z  TranslationStandardOffset=0  TranslationCartesianOffset=smiData.RigidTransform(477).translation  TranslationROffset=0  TranslationROffsetUnits=m  TranslationZOffset=0  TranslationZOffsetUnits=m  TranslationThetaOffset=0  TranslationThetaOffsetUnits=deg  RotationMethod=ArbitraryAxis  RotationAngleUnits=rad  RotationStandardAxis=+Z  RotationAngle=smiData.RigidTransform(477).angle  RotationArbitraryAxis=smiData.RigidTransform(477).axis  FollAlignAxisA=+X  BaseAlignAxisA=+Y  FollAlignAxisB=+Y  BaseAlignAxisB=+Z  RotationSequenceAxes=FollowerAxes  RotationSequence=XYX  RotationSequenceAngles=[0 0 0]  RotationSequenceAnglesUnits=deg  RotationMatrix=[1 0 0; 0 1 0; 0 0 1]
  Transform51 : sm_lib/Frames and Transforms/Rigid Transform  TranslationMethod=Cartesian  TranslationLengthUnit=in  TranslationStandardAxis=+Z  TranslationStandardOffset=0  TranslationCartesianOffset=smiData.RigidTransform(478).translation  TranslationROffset=0  TranslationROffsetUnits=m  TranslationZOffset=0  TranslationZOffsetUnits=m  TranslationThetaOffset=0  TranslationThetaOffsetUnits=deg  RotationMethod=ArbitraryAxis  RotationAngleUnits=rad  RotationStandardAxis=+Z  RotationAngle=smiData.RigidTransform(478).angle  RotationArbitraryAxis=smiData.RigidTransform(478).axis  FollAlignAxisA=+X  BaseAlignAxisA=+Y  FollAlignAxisB=+Y  BaseAlignAxisB=+Z  RotationSequenceAxes=FollowerAxes  RotationSequence=XYX  RotationSequenceAngles=[0 0 0]  RotationSequenceAnglesUnits=deg  RotationMatrix=[1 0 0; 0 1 0; 0 0 1]
  Transform52 : sm_lib/Frames and Transforms/Rigid Transform  TranslationMethod=Cartesian  TranslationLengthUnit=in  TranslationStandardAxis=+Z  TranslationStandardOffset=0  TranslationCartesianOffset=smiData.RigidTransform(479).translation  TranslationROffset=0  TranslationROffsetUnits=m  TranslationZOffset=0  TranslationZOffsetUnits=m  TranslationThetaOffset=0  TranslationThetaOffsetUnits=deg  RotationMethod=ArbitraryAxis  RotationAngleUnits=rad  RotationStandardAxis=+Z  RotationAngle=smiData.RigidTransform(479).angle  RotationArbitraryAxis=smiData.RigidTransform(479).axis  FollAlignAxisA=+X  BaseAlignAxisA=+Y  FollAlignAxisB=+Y  BaseAlignAxisB=+Z  RotationSequenceAxes=FollowerAxes  RotationSequence=XYX  RotationSequenceAngles=[0 0 0]  RotationSequenceAnglesUnits=deg  RotationMatrix=[1 0 0; 0 1 0; 0 0 1]
  Transform53 : sm_lib/Frames and Transforms/Rigid Transform  TranslationMethod=Cartesian  TranslationLengthUnit=in  TranslationStandardAxis=+Z  TranslationStandardOffset=0  TranslationCartesianOffset=smiData.RigidTransform(480).translation  TranslationROffset=0  TranslationROffsetUnits=m  TranslationZOffset=0  TranslationZOffsetUnits=m  TranslationThetaOffset=0  TranslationThetaOffsetUnits=deg  RotationMethod=ArbitraryAxis  RotationAngleUnits=rad  RotationStandardAxis=+Z  RotationAngle=smiData.RigidTransform(480).angle  RotationArbitraryAxis=smiData.RigidTransform(480).axis  FollAlignAxisA=+X  BaseAlignAxisA=+Y  FollAlignAxisB=+Y  BaseAlignAxisB=+Z  RotationSequenceAxes=FollowerAxes  RotationSequence=XYX  RotationSequenceAngles=[0 0 0]  RotationSequenceAnglesUnits=deg  RotationMatrix=[1 0 0; 0 1 0; 0 0 1]
  Transform54 : sm_lib/Frames and Transforms/Rigid Transform  TranslationMethod=Cartesian  TranslationLengthUnit=in  TranslationStandardAxis=+Z  TranslationStandardOffset=0  TranslationCartesianOffset=smiData.RigidTransform(481).translation  TranslationROffset=0  TranslationROffsetUnits=m  TranslationZOffset=0  TranslationZOffsetUnits=m  TranslationThetaOffset=0  TranslationThetaOffsetUnits=deg  RotationMethod=ArbitraryAxis  RotationAngleUnits=rad  RotationStandardAxis=+Z  RotationAngle=smiData.RigidTransform(481).angle  RotationArbitraryAxis=smiData.RigidTransform(481).axis  FollAlignAxisA=+X  BaseAlignAxisA=+Y  FollAlignAxisB=+Y  BaseAlignAxisB=+Z  RotationSequenceAxes=FollowerAxes  RotationSequence=XYX  RotationSequenceAngles=[0 0 0]  RotationSequenceAnglesUnits=deg  RotationMatrix=[1 0 0; 0 1 0; 0 0 1]
  Transform55 : sm_lib/Frames and Transforms/Rigid Transform  TranslationMethod=Cartesian  TranslationLengthUnit=in  TranslationStandardAxis=+Z  TranslationStandardOffset=0  TranslationCartesianOffset=smiData.RigidTransform(482).translation  TranslationROffset=0  TranslationROffsetUnits=m  TranslationZOffset=0  TranslationZOffsetUnits=m  TranslationThetaOffset=0  TranslationThetaOffsetUnits=deg  RotationMethod=ArbitraryAxis  RotationAngleUnits=rad  RotationStandardAxis=+Z  RotationAngle=smiData.RigidTransform(482).angle  RotationArbitraryAxis=smiData.RigidTransform(482).axis  FollAlignAxisA=+X  BaseAlignAxisA=+Y  FollAlignAxisB=+Y  BaseAlignAxisB=+Z  RotationSequenceAxes=FollowerAxes  RotationSequence=XYX  RotationSequenceAngles=[0 0 0]  RotationSequenceAnglesUnits=deg  RotationMatrix=[1 0 0; 0 1 0; 0 0 1]
  Transform56 : sm_lib/Frames and Transforms/Rigid Transform  TranslationMethod=Cartesian  TranslationLengthUnit=in  TranslationStandardAxis=+Z  TranslationStandardOffset=0  TranslationCartesianOffset=smiData.RigidTransform(483).translation  TranslationROffset=0  TranslationROffsetUnits=m  TranslationZOffset=0  TranslationZOffsetUnits=m  TranslationThetaOffset=0  TranslationThetaOffsetUnits=deg  RotationMethod=ArbitraryAxis  RotationAngleUnits=rad  RotationStandardAxis=+Z  RotationAngle=smiData.RigidTransform(483).angle  RotationArbitraryAxis=smiData.RigidTransform(483).axis  FollAlignAxisA=+X  BaseAlignAxisA=+Y  FollAlignAxisB=+Y  BaseAlignAxisB=+Z  RotationSequenceAxes=FollowerAxes  RotationSequence=XYX  RotationSequenceAngles=[0 0 0]  RotationSequenceAnglesUnits=deg  RotationMatrix=[1 0 0; 0 1 0; 0 0 1]
  Transform57 : sm_lib/Frames and Transforms/Rigid Transform  TranslationMethod=Cartesian  TranslationLengthUnit=in  TranslationStandardAxis=+Z  TranslationStandardOffset=0  TranslationCartesianOffset=smiData.RigidTransform(484).translation  TranslationROffset=0  TranslationROffsetUnits=m  TranslationZOffset=0  TranslationZOffsetUnits=m  TranslationThetaOffset=0  TranslationThetaOffsetUnits=deg  RotationMethod=ArbitraryAxis  RotationAngleUnits=rad  RotationStandardAxis=+Z  RotationAngle=smiData.RigidTransform(484).angle  RotationArbitraryAxis=smiData.RigidTransform(484).axis  FollAlignAxisA=+X  BaseAlignAxisA=+Y  FollAlignAxisB=+Y  BaseAlignAxisB=+Z  RotationSequenceAxes=FollowerAxes  RotationSequence=XYX  RotationSequenceAngles=[0 0 0]  RotationSequenceAnglesUnits=deg  RotationMatrix=[1 0 0; 0 1 0; 0 0 1]
  Transform58 : sm_lib/Frames and Transforms/Rigid Transform  TranslationMethod=Cartesian  TranslationLengthUnit=in  TranslationStandardAxis=+Z  TranslationStandardOffset=0  TranslationCartesianOffset=smiData.RigidTransform(485).translation  TranslationROffset=0  TranslationROffsetUnits=m  TranslationZOffset=0  TranslationZOffsetUnits=m  TranslationThetaOffset=0  TranslationThetaOffsetUnits=deg  RotationMethod=ArbitraryAxis  RotationAngleUnits=rad  RotationStandardAxis=+Z  RotationAngle=smiData.RigidTransform(485).angle  RotationArbitraryAxis=smiData.RigidTransform(485).axis  FollAlignAxisA=+X  BaseAlignAxisA=+Y  FollAlignAxisB=+Y  BaseAlignAxisB=+Z  RotationSequenceAxes=FollowerAxes  RotationSequence=XYX  RotationSequenceAngles=[0 0 0]  RotationSequenceAnglesUnits=deg  RotationMatrix=[1 0 0; 0 1 0; 0 0 1]
  Transform59 : sm_lib/Frames and Transforms/Rigid Transform  TranslationMethod=Cartesian  TranslationLengthUnit=in  TranslationStandardAxis=+Z  TranslationStandardOffset=0  TranslationCartesianOffset=smiData.RigidTransform(486).translation  TranslationROffset=0  TranslationROffsetUnits=m  TranslationZOffset=0  TranslationZOffsetUnits=m  TranslationThetaOffset=0  TranslationThetaOffsetUnits=deg  RotationMethod=ArbitraryAxis  RotationAngleUnits=rad  RotationStandardAxis=+Z  RotationAngle=smiData.RigidTransform(486).angle  RotationArbitraryAxis=smiData.RigidTransform(486).axis  FollAlignAxisA=+X  BaseAlignAxisA=+Y  FollAlignAxisB=+Y  BaseAlignAxisB=+Z  RotationSequenceAxes=FollowerAxes  RotationSequence=XYX  RotationSequenceAngles=[0 0 0]  RotationSequenceAnglesUnits=deg  RotationMatrix=[1 0 0; 0 1 0; 0 0 1]
  Transform6 : sm_lib/Frames and Transforms/Rigid Transform  TranslationMethod=Cartesian  TranslationLengthUnit=in  TranslationStandardAxis=+Z  TranslationStandardOffset=0  TranslationCartesianOffset=smiData.RigidTransform(433).translation  TranslationROffset=0  TranslationROffsetUnits=m  TranslationZOffset=0  TranslationZOffsetUnits=m  TranslationThetaOffset=0  TranslationThetaOffsetUnits=deg  RotationMethod=ArbitraryAxis  RotationAngleUnits=rad  RotationStandardAxis=+Z  RotationAngle=smiData.RigidTransform(433).angle  RotationArbitraryAxis=smiData.RigidTransform(433).axis  FollAlignAxisA=+X  BaseAlignAxisA=+Y  FollAlignAxisB=+Y  BaseAlignAxisB=+Z  RotationSequenceAxes=FollowerAxes  RotationSequence=XYX  RotationSequenceAngles=[0 0 0]  RotationSequenceAnglesUnits=deg  RotationMatrix=[1 0 0; 0 1 0; 0 0 1]
  Transform60 : sm_lib/Frames and Transforms/Rigid Transform  TranslationMethod=Cartesian  TranslationLengthUnit=in  TranslationStandardAxis=+Z  TranslationStandardOffset=0  TranslationCartesianOffset=smiData.RigidTransform(487).translation  TranslationROffset=0  TranslationROffsetUnits=m  TranslationZOffset=0  TranslationZOffsetUnits=m  TranslationThetaOffset=0  TranslationThetaOffsetUnits=deg  RotationMethod=ArbitraryAxis  RotationAngleUnits=rad  RotationStandardAxis=+Z  RotationAngle=smiData.RigidTransform(487).angle  RotationArbitraryAxis=smiData.RigidTransform(487).axis  FollAlignAxisA=+X  BaseAlignAxisA=+Y  FollAlignAxisB=+Y  BaseAlignAxisB=+Z  RotationSequenceAxes=FollowerAxes  RotationSequence=XYX  RotationSequenceAngles=[0 0 0]  RotationSequenceAnglesUnits=deg  RotationMatrix=[1 0 0; 0 1 0; 0 0 1]
  Transform61 : sm_lib/Frames and Transforms/Rigid Transform  TranslationMethod=Cartesian  TranslationLengthUnit=in  TranslationStandardAxis=+Z  TranslationStandardOffset=0  TranslationCartesianOffset=smiData.RigidTransform(488).translation  TranslationROffset=0  TranslationROffsetUnits=m  TranslationZOffset=0  TranslationZOffsetUnits=m  TranslationThetaOffset=0  TranslationThetaOffsetUnits=deg  RotationMethod=ArbitraryAxis  RotationAngleUnits=rad  RotationStandardAxis=+Z  RotationAngle=smiData.RigidTransform(488).angle  RotationArbitraryAxis=smiData.RigidTransform(488).axis  FollAlignAxisA=+X  BaseAlignAxisA=+Y  FollAlignAxisB=+Y  BaseAlignAxisB=+Z  RotationSequenceAxes=FollowerAxes  RotationSequence=XYX  RotationSequenceAngles=[0 0 0]  RotationSequenceAnglesUnits=deg  RotationMatrix=[1 0 0; 0 1 0; 0 0 1]
  Transform62 : sm_lib/Frames and Transforms/Rigid Transform  TranslationMethod=Cartesian  TranslationLengthUnit=in  TranslationStandardAxis=+Z  TranslationStandardOffset=0  TranslationCartesianOffset=smiData.RigidTransform(489).translation  TranslationROffset=0  TranslationROffsetUnits=m  TranslationZOffset=0  TranslationZOffsetUnits=m  TranslationThetaOffset=0  TranslationThetaOffsetUnits=deg  RotationMethod=ArbitraryAxis  RotationAngleUnits=rad  RotationStandardAxis=+Z  RotationAngle=smiData.RigidTransform(489).angle  RotationArbitraryAxis=smiData.RigidTransform(489).axis  FollAlignAxisA=+X  BaseAlignAxisA=+Y  FollAlignAxisB=+Y  BaseAlignAxisB=+Z  RotationSequenceAxes=FollowerAxes  RotationSequence=XYX  RotationSequenceAngles=[0 0 0]  RotationSequenceAnglesUnits=deg  RotationMatrix=[1 0 0; 0 1 0; 0 0 1]
  Transform63 : sm_lib/Frames and Transforms/Rigid Transform  TranslationMethod=Cartesian  TranslationLengthUnit=in  TranslationStandardAxis=+Z  TranslationStandardOffset=0  TranslationCartesianOffset=smiData.RigidTransform(490).translation  TranslationROffset=0  TranslationROffsetUnits=m  TranslationZOffset=0  TranslationZOffsetUnits=m  TranslationThetaOffset=0  TranslationThetaOffsetUnits=deg  RotationMethod=ArbitraryAxis  RotationAngleUnits=rad  RotationStandardAxis=+Z  RotationAngle=smiData.RigidTransform(490).angle  RotationArbitraryAxis=smiData.RigidTransform(490).axis  FollAlignAxisA=+X  BaseAlignAxisA=+Y  FollAlignAxisB=+Y  BaseAlignAxisB=+Z  RotationSequenceAxes=FollowerAxes  RotationSequence=XYX  RotationSequenceAngles=[0 0 0]  RotationSequenceAnglesUnits=deg  RotationMatrix=[1 0 0; 0 1 0; 0 0 1]
  Transform64 : sm_lib/Frames and Transforms/Rigid Transform  TranslationMethod=Cartesian  TranslationLengthUnit=in  TranslationStandardAxis=+Z  TranslationStandardOffset=0  TranslationCartesianOffset=smiData.RigidTransform(491).translation  TranslationROffset=0  TranslationROffsetUnits=m  TranslationZOffset=0  TranslationZOffsetUnits=m  TranslationThetaOffset=0  TranslationThetaOffsetUnits=deg  RotationMethod=ArbitraryAxis  RotationAngleUnits=rad  RotationStandardAxis=+Z  RotationAngle=smiData.RigidTransform(491).angle  RotationArbitraryAxis=smiData.RigidTransform(491).axis  FollAlignAxisA=+X  BaseAlignAxisA=+Y  FollAlignAxisB=+Y  BaseAlignAxisB=+Z  RotationSequenceAxes=FollowerAxes  RotationSequence=XYX  RotationSequenceAngles=[0 0 0]  RotationSequenceAnglesUnits=deg  RotationMatrix=[1 0 0; 0 1 0; 0 0 1]
  Transform65 : sm_lib/Frames and Transforms/Rigid Transform  TranslationMethod=Cartesian  TranslationLengthUnit=in  TranslationStandardAxis=+Z  TranslationStandardOffset=0  TranslationCartesianOffset=smiData.RigidTransform(492).translation  TranslationROffset=0  TranslationROffsetUnits=m  TranslationZOffset=0  TranslationZOffsetUnits=m  TranslationThetaOffset=0  TranslationThetaOffsetUnits=deg  RotationMethod=ArbitraryAxis  RotationAngleUnits=rad  RotationStandardAxis=+Z  RotationAngle=smiData.RigidTransform(492).angle  RotationArbitraryAxis=smiData.RigidTransform(492).axis  FollAlignAxisA=+X  BaseAlignAxisA=+Y  FollAlignAxisB=+Y  BaseAlignAxisB=+Z  RotationSequenceAxes=FollowerAxes  RotationSequence=XYX  RotationSequenceAngles=[0 0 0]  RotationSequenceAnglesUnits=deg  RotationMatrix=[1 0 0; 0 1 0; 0 0 1]
  Transform66 : sm_lib/Frames and Transforms/Rigid Transform  TranslationMethod=Cartesian  TranslationLengthUnit=in  TranslationStandardAxis=+Z  TranslationStandardOffset=0  TranslationCartesianOffset=smiData.RigidTransform(493).translation  TranslationROffset=0  TranslationROffsetUnits=m  TranslationZOffset=0  TranslationZOffsetUnits=m  TranslationThetaOffset=0  TranslationThetaOffsetUnits=deg  RotationMethod=ArbitraryAxis  RotationAngleUnits=rad  RotationStandardAxis=+Z  RotationAngle=smiData.RigidTransform(493).angle  RotationArbitraryAxis=smiData.RigidTransform(493).axis  FollAlignAxisA=+X  BaseAlignAxisA=+Y  FollAlignAxisB=+Y  BaseAlignAxisB=+Z  RotationSequenceAxes=FollowerAxes  RotationSequence=XYX  RotationSequenceAngles=[0 0 0]  RotationSequenceAnglesUnits=deg  RotationMatrix=[1 0 0; 0 1 0; 0 0 1]
  Transform67 : sm_lib/Frames and Transforms/Rigid Transform  TranslationMethod=Cartesian  TranslationLengthUnit=in  TranslationStandardAxis=+Z  TranslationStandardOffset=0  TranslationCartesianOffset=smiData.RigidTransform(494).translation  TranslationROffset=0  TranslationROffsetUnits=m  TranslationZOffset=0  TranslationZOffsetUnits=m  TranslationThetaOffset=0  TranslationThetaOffsetUnits=deg  RotationMethod=ArbitraryAxis  RotationAngleUnits=rad  RotationStandardAxis=+Z  RotationAngle=smiData.RigidTransform(494).angle  RotationArbitraryAxis=smiData.RigidTransform(494).axis  FollAlignAxisA=+X  BaseAlignAxisA=+Y  FollAlignAxisB=+Y  BaseAlignAxisB=+Z  RotationSequenceAxes=FollowerAxes  RotationSequence=XYX  RotationSequenceAngles=[0 0 0]  RotationSequenceAnglesUnits=deg  RotationMatrix=[1 0 0; 0 1 0; 0 0 1]
  Transform68 : sm_lib/Frames and Transforms/Rigid Transform  TranslationMethod=Cartesian  TranslationLengthUnit=in  TranslationStandardAxis=+Z  TranslationStandardOffset=0  TranslationCartesianOffset=smiData.RigidTransform(495).translation  TranslationROffset=0  TranslationROffsetUnits=m  TranslationZOffset=0  TranslationZOffsetUnits=m  TranslationThetaOffset=0  TranslationThetaOffsetUnits=deg  RotationMethod=ArbitraryAxis  RotationAngleUnits=rad  RotationStandardAxis=+Z  RotationAngle=smiData.RigidTransform(495).angle  RotationArbitraryAxis=smiData.RigidTransform(495).axis  FollAlignAxisA=+X  BaseAlignAxisA=+Y  FollAlignAxisB=+Y  BaseAlignAxisB=+Z  RotationSequenceAxes=FollowerAxes  RotationSequence=XYX  RotationSequenceAngles=[0 0 0]  RotationSequenceAnglesUnits=deg  RotationMatrix=[1 0 0; 0 1 0; 0 0 1]
  Transform69 : sm_lib/Frames and Transforms/Rigid Transform  TranslationMethod=Cartesian  TranslationLengthUnit=in  TranslationStandardAxis=+Z  TranslationStandardOffset=0  TranslationCartesianOffset=smiData.RigidTransform(496).translation  TranslationROffset=0  TranslationROffsetUnits=m  TranslationZOffset=0  TranslationZOffsetUnits=m  TranslationThetaOffset=0  TranslationThetaOffsetUnits=deg  RotationMethod=ArbitraryAxis  RotationAngleUnits=rad  RotationStandardAxis=+Z  RotationAngle=smiData.RigidTransform(496).angle  RotationArbitraryAxis=smiData.RigidTransform(496).axis  FollAlignAxisA=+X  BaseAlignAxisA=+Y  FollAlignAxisB=+Y  BaseAlignAxisB=+Z  RotationSequenceAxes=FollowerAxes  RotationSequence=XYX  RotationSequenceAngles=[0 0 0]  RotationSequenceAnglesUnits=deg  RotationMatrix=[1 0 0; 0 1 0; 0 0 1]
  Transform7 : sm_lib/Frames and Transforms/Rigid Transform  TranslationMethod=Cartesian  TranslationLengthUnit=in  TranslationStandardAxis=+Z  TranslationStandardOffset=0  TranslationCartesianOffset=smiData.RigidTransform(434).translation  TranslationROffset=0  TranslationROffsetUnits=m  TranslationZOffset=0  TranslationZOffsetUnits=m  TranslationThetaOffset=0  TranslationThetaOffsetUnits=deg  RotationMethod=ArbitraryAxis  RotationAngleUnits=rad  RotationStandardAxis=+Z  RotationAngle=smiData.RigidTransform(434).angle  RotationArbitraryAxis=smiData.RigidTransform(434).axis  FollAlignAxisA=+X  BaseAlignAxisA=+Y  FollAlignAxisB=+Y  BaseAlignAxisB=+Z  RotationSequenceAxes=FollowerAxes  RotationSequence=XYX  RotationSequenceAngles=[0 0 0]  RotationSequenceAnglesUnits=deg  RotationMatrix=[1 0 0; 0 1 0; 0 0 1]
  Transform70 : sm_lib/Frames and Transforms/Rigid Transform  TranslationMethod=Cartesian  TranslationLengthUnit=in  TranslationStandardAxis=+Z  TranslationStandardOffset=0  TranslationCartesianOffset=smiData.RigidTransform(497).translation  TranslationROffset=0  TranslationROffsetUnits=m  TranslationZOffset=0  TranslationZOffsetUnits=m  TranslationThetaOffset=0  TranslationThetaOffsetUnits=deg  RotationMethod=ArbitraryAxis  RotationAngleUnits=rad  RotationStandardAxis=+Z  RotationAngle=smiData.RigidTransform(497).angle  RotationArbitraryAxis=smiData.RigidTransform(497).axis  FollAlignAxisA=+X  BaseAlignAxisA=+Y  FollAlignAxisB=+Y  BaseAlignAxisB=+Z  RotationSequenceAxes=FollowerAxes  RotationSequence=XYX  RotationSequenceAngles=[0 0 0]  RotationSequenceAnglesUnits=deg  RotationMatrix=[1 0 0; 0 1 0; 0 0 1]
  Transform71 : sm_lib/Frames and Transforms/Rigid Transform  TranslationMethod=Cartesian  TranslationLengthUnit=in  TranslationStandardAxis=+Z  TranslationStandardOffset=0  TranslationCartesianOffset=smiData.RigidTransform(498).translation  TranslationROffset=0  TranslationROffsetUnits=m  TranslationZOffset=0  TranslationZOffsetUnits=m  TranslationThetaOffset=0  TranslationThetaOffsetUnits=deg  RotationMethod=ArbitraryAxis  RotationAngleUnits=rad  RotationStandardAxis=+Z  RotationAngle=smiData.RigidTransform(498).angle  RotationArbitraryAxis=smiData.RigidTransform(498).axis  FollAlignAxisA=+X  BaseAlignAxisA=+Y  FollAlignAxisB=+Y  BaseAlignAxisB=+Z  RotationSequenceAxes=FollowerAxes  RotationSequence=XYX  RotationSequenceAngles=[0 0 0]  RotationSequenceAnglesUnits=deg  RotationMatrix=[1 0 0; 0 1 0; 0 0 1]
  Transform72 : sm_lib/Frames and Transforms/Rigid Transform  TranslationMethod=Cartesian  TranslationLengthUnit=in  TranslationStandardAxis=+Z  TranslationStandardOffset=0  TranslationCartesianOffset=smiData.RigidTransform(499).translation  TranslationROffset=0  TranslationROffsetUnits=m  TranslationZOffset=0  TranslationZOffsetUnits=m  TranslationThetaOffset=0  TranslationThetaOffsetUnits=deg  RotationMethod=ArbitraryAxis  RotationAngleUnits=rad  RotationStandardAxis=+Z  RotationAngle=smiData.RigidTransform(499).angle  RotationArbitraryAxis=smiData.RigidTransform(499).axis  FollAlignAxisA=+X  BaseAlignAxisA=+Y  FollAlignAxisB=+Y  BaseAlignAxisB=+Z  RotationSequenceAxes=FollowerAxes  RotationSequence=XYX  RotationSequenceAngles=[0 0 0]  RotationSequenceAnglesUnits=deg  RotationMatrix=[1 0 0; 0 1 0; 0 0 1]
  Transform73 : sm_lib/Frames and Transforms/Rigid Transform  TranslationMethod=Cartesian  TranslationLengthUnit=in  TranslationStandardAxis=+Z  TranslationStandardOffset=0  TranslationCartesianOffset=smiData.RigidTransform(500).translation  TranslationROffset=0  TranslationROffsetUnits=m  TranslationZOffset=0  TranslationZOffsetUnits=m  TranslationThetaOffset=0  TranslationThetaOffsetUnits=deg  RotationMethod=ArbitraryAxis  RotationAngleUnits=rad  RotationStandardAxis=+Z  RotationAngle=smiData.RigidTransform(500).angle  RotationArbitraryAxis=smiData.RigidTransform(500).axis  FollAlignAxisA=+X  BaseAlignAxisA=+Y  FollAlignAxisB=+Y  BaseAlignAxisB=+Z  RotationSequenceAxes=FollowerAxes  RotationSequence=XYX  RotationSequenceAngles=[0 0 0]  RotationSequenceAnglesUnits=deg  RotationMatrix=[1 0 0; 0 1 0; 0 0 1]
  Transform74 : sm_lib/Frames and Transforms/Rigid Transform  TranslationMethod=Cartesian  TranslationLengthUnit=in  TranslationStandardAxis=+Z  TranslationStandardOffset=0  TranslationCartesianOffset=smiData.RigidTransform(501).translation  TranslationROffset=0  TranslationROffsetUnits=m  TranslationZOffset=0  TranslationZOffsetUnits=m  TranslationThetaOffset=0  TranslationThetaOffsetUnits=deg  RotationMethod=ArbitraryAxis  RotationAngleUnits=rad  RotationStandardAxis=+Z  RotationAngle=smiData.RigidTransform(501).angle  RotationArbitraryAxis=smiData.RigidTransform(501).axis  FollAlignAxisA=+X  BaseAlignAxisA=+Y  FollAlignAxisB=+Y  BaseAlignAxisB=+Z  RotationSequenceAxes=FollowerAxes  RotationSequence=XYX  RotationSequenceAngles=[0 0 0]  RotationSequenceAnglesUnits=deg  RotationMatrix=[1 0 0; 0 1 0; 0 0 1]
  Transform75 : sm_lib/Frames and Transforms/Rigid Transform  TranslationMethod=Cartesian  TranslationLengthUnit=in  TranslationStandardAxis=+Z  TranslationStandardOffset=0  TranslationCartesianOffset=smiData.RigidTransform(502).translation  TranslationROffset=0  TranslationROffsetUnits=m  TranslationZOffset=0  TranslationZOffsetUnits=m  TranslationThetaOffset=0  TranslationThetaOffsetUnits=deg  RotationMethod=ArbitraryAxis  RotationAngleUnits=rad  RotationStandardAxis=+Z  RotationAngle=smiData.RigidTransform(502).angle  RotationArbitraryAxis=smiData.RigidTransform(502).axis  FollAlignAxisA=+X  BaseAlignAxisA=+Y  FollAlignAxisB=+Y  BaseAlignAxisB=+Z  RotationSequenceAxes=FollowerAxes  RotationSequence=XYX  RotationSequenceAngles=[0 0 0]  RotationSequenceAnglesUnits=deg  RotationMatrix=[1 0 0; 0 1 0; 0 0 1]
  Transform76 : sm_lib/Frames and Transforms/Rigid Transform  TranslationMethod=Cartesian  TranslationLengthUnit=in  TranslationStandardAxis=+Z  TranslationStandardOffset=0  TranslationCartesianOffset=smiData.RigidTransform(503).translation  TranslationROffset=0  TranslationROffsetUnits=m  TranslationZOffset=0  TranslationZOffsetUnits=m  TranslationThetaOffset=0  TranslationThetaOffsetUnits=deg  RotationMethod=ArbitraryAxis  RotationAngleUnits=rad  RotationStandardAxis=+Z  RotationAngle=smiData.RigidTransform(503).angle  RotationArbitraryAxis=smiData.RigidTransform(503).axis  FollAlignAxisA=+X  BaseAlignAxisA=+Y  FollAlignAxisB=+Y  BaseAlignAxisB=+Z  RotationSequenceAxes=FollowerAxes  RotationSequence=XYX  RotationSequenceAngles=[0 0 0]  RotationSequenceAnglesUnits=deg  RotationMatrix=[1 0 0; 0 1 0; 0 0 1]
  Transform77 : sm_lib/Frames and Transforms/Rigid Transform  TranslationMethod=Cartesian  TranslationLengthUnit=in  TranslationStandardAxis=+Z  TranslationStandardOffset=0  TranslationCartesianOffset=smiData.RigidTransform(504).translation  TranslationROffset=0  TranslationROffsetUnits=m  TranslationZOffset=0  TranslationZOffsetUnits=m  TranslationThetaOffset=0  TranslationThetaOffsetUnits=deg  RotationMethod=ArbitraryAxis  RotationAngleUnits=rad  RotationStandardAxis=+Z  RotationAngle=smiData.RigidTransform(504).angle  RotationArbitraryAxis=smiData.RigidTransform(504).axis  FollAlignAxisA=+X  BaseAlignAxisA=+Y  FollAlignAxisB=+Y  BaseAlignAxisB=+Z  RotationSequenceAxes=FollowerAxes  RotationSequence=XYX  RotationSequenceAngles=[0 0 0]  RotationSequenceAnglesUnits=deg  RotationMatrix=[1 0 0; 0 1 0; 0 0 1]
  Transform78 : sm_lib/Frames and Transforms/Rigid Transform  TranslationMethod=Cartesian  TranslationLengthUnit=in  TranslationStandardAxis=+Z  TranslationStandardOffset=0  TranslationCartesianOffset=smiData.RigidTransform(505).translation  TranslationROffset=0  TranslationROffsetUnits=m  TranslationZOffset=0  TranslationZOffsetUnits=m  TranslationThetaOffset=0  TranslationThetaOffsetUnits=deg  RotationMethod=ArbitraryAxis  RotationAngleUnits=rad  RotationStandardAxis=+Z  RotationAngle=smiData.RigidTransform(505).angle  RotationArbitraryAxis=smiData.RigidTransform(505).axis  FollAlignAxisA=+X  BaseAlignAxisA=+Y  FollAlignAxisB=+Y  BaseAlignAxisB=+Z  RotationSequenceAxes=FollowerAxes  RotationSequence=XYX  RotationSequenceAngles=[0 0 0]  RotationSequenceAnglesUnits=deg  RotationMatrix=[1 0 0; 0 1 0; 0 0 1]
  Transform79 : sm_lib/Frames and Transforms/Rigid Transform  TranslationMethod=Cartesian  TranslationLengthUnit=in  TranslationStandardAxis=+Z  TranslationStandardOffset=0  TranslationCartesianOffset=smiData.RigidTransform(506).translation  TranslationROffset=0  TranslationROffsetUnits=m  TranslationZOffset=0  TranslationZOffsetUnits=m  TranslationThetaOffset=0  TranslationThetaOffsetUnits=deg  RotationMethod=ArbitraryAxis  RotationAngleUnits=rad  RotationStandardAxis=+Z  RotationAngle=smiData.RigidTransform(506).angle  RotationArbitraryAxis=smiData.RigidTransform(506).axis  FollAlignAxisA=+X  BaseAlignAxisA=+Y  FollAlignAxisB=+Y  BaseAlignAxisB=+Z  RotationSequenceAxes=FollowerAxes  RotationSequence=XYX  RotationSequenceAngles=[0 0 0]  RotationSequenceAnglesUnits=deg  RotationMatrix=[1 0 0; 0 1 0; 0 0 1]
  Transform8 : sm_lib/Frames and Transforms/Rigid Transform  TranslationMethod=Cartesian  TranslationLengthUnit=in  TranslationStandardAxis=+Z  TranslationStandardOffset=0  TranslationCartesianOffset=smiData.RigidTransform(435).translation  TranslationROffset=0  TranslationROffsetUnits=m  TranslationZOffset=0  TranslationZOffsetUnits=m  TranslationThetaOffset=0  TranslationThetaOffsetUnits=deg  RotationMethod=ArbitraryAxis  RotationAngleUnits=rad  RotationStandardAxis=+Z  RotationAngle=smiData.RigidTransform(435).angle  RotationArbitraryAxis=smiData.RigidTransform(435).axis  FollAlignAxisA=+X  BaseAlignAxisA=+Y  FollAlignAxisB=+Y  BaseAlignAxisB=+Z  RotationSequenceAxes=FollowerAxes  RotationSequence=XYX  RotationSequenceAngles=[0 0 0]  RotationSequenceAnglesUnits=deg  RotationMatrix=[1 0 0; 0 1 0; 0 0 1]
  Transform80 : sm_lib/Frames and Transforms/Rigid Transform  TranslationMethod=Cartesian  TranslationLengthUnit=in  TranslationStandardAxis=+Z  TranslationStandardOffset=0  TranslationCartesianOffset=smiData.RigidTransform(507).translation  TranslationROffset=0  TranslationROffsetUnits=m  TranslationZOffset=0  TranslationZOffsetUnits=m  TranslationThetaOffset=0  TranslationThetaOffsetUnits=deg  RotationMethod=ArbitraryAxis  RotationAngleUnits=rad  RotationStandardAxis=+Z  RotationAngle=smiData.RigidTransform(507).angle  RotationArbitraryAxis=smiData.RigidTransform(507).axis  FollAlignAxisA=+X  BaseAlignAxisA=+Y  FollAlignAxisB=+Y  BaseAlignAxisB=+Z  RotationSequenceAxes=FollowerAxes  RotationSequence=XYX  RotationSequenceAngles=[0 0 0]  RotationSequenceAnglesUnits=deg  RotationMatrix=[1 0 0; 0 1 0; 0 0 1]
  Transform81 : sm_lib/Frames and Transforms/Rigid Transform  TranslationMethod=Cartesian  TranslationLengthUnit=in  TranslationStandardAxis=+Z  TranslationStandardOffset=0  TranslationCartesianOffset=smiData.RigidTransform(508).translation  TranslationROffset=0  TranslationROffsetUnits=m  TranslationZOffset=0  TranslationZOffsetUnits=m  TranslationThetaOffset=0  TranslationThetaOffsetUnits=deg  RotationMethod=ArbitraryAxis  RotationAngleUnits=rad  RotationStandardAxis=+Z  RotationAngle=smiData.RigidTransform(508).angle  RotationArbitraryAxis=smiData.RigidTransform(508).axis  FollAlignAxisA=+X  BaseAlignAxisA=+Y  FollAlignAxisB=+Y  BaseAlignAxisB=+Z  RotationSequenceAxes=FollowerAxes  RotationSequence=XYX  RotationSequenceAngles=[0 0 0]  RotationSequenceAnglesUnits=deg  RotationMatrix=[1 0 0; 0 1 0; 0 0 1]
  Transform82 : sm_lib/Frames and Transforms/Rigid Transform  TranslationMethod=Cartesian  TranslationLengthUnit=in  TranslationStandardAxis=+Z  TranslationStandardOffset=0  TranslationCartesianOffset=smiData.RigidTransform(509).translation  TranslationROffset=0  TranslationROffsetUnits=m  TranslationZOffset=0  TranslationZOffsetUnits=m  TranslationThetaOffset=0  TranslationThetaOffsetUnits=deg  RotationMethod=ArbitraryAxis  RotationAngleUnits=rad  RotationStandardAxis=+Z  RotationAngle=smiData.RigidTransform(509).angle  RotationArbitraryAxis=smiData.RigidTransform(509).axis  FollAlignAxisA=+X  BaseAlignAxisA=+Y  FollAlignAxisB=+Y  BaseAlignAxisB=+Z  RotationSequenceAxes=FollowerAxes  RotationSequence=XYX  RotationSequenceAngles=[0 0 0]  RotationSequenceAnglesUnits=deg  RotationMatrix=[1 0 0; 0 1 0; 0 0 1]
  Transform83 : sm_lib/Frames and Transforms/Rigid Transform  TranslationMethod=Cartesian  TranslationLengthUnit=in  TranslationStandardAxis=+Z  TranslationStandardOffset=0  TranslationCartesianOffset=smiData.RigidTransform(510).translation  TranslationROffset=0  TranslationROffsetUnits=m  TranslationZOffset=0  TranslationZOffsetUnits=m  TranslationThetaOffset=0  TranslationThetaOffsetUnits=deg  RotationMethod=ArbitraryAxis  RotationAngleUnits=rad  RotationStandardAxis=+Z  RotationAngle=smiData.RigidTransform(510).angle  RotationArbitraryAxis=smiData.RigidTransform(510).axis  FollAlignAxisA=+X  BaseAlignAxisA=+Y  FollAlignAxisB=+Y  BaseAlignAxisB=+Z  RotationSequenceAxes=FollowerAxes  RotationSequence=XYX  RotationSequenceAngles=[0 0 0]  RotationSequenceAnglesUnits=deg  RotationMatrix=[1 0 0; 0 1 0; 0 0 1]
  Transform84 : sm_lib/Frames and Transforms/Rigid Transform  TranslationMethod=Cartesian  TranslationLengthUnit=in  TranslationStandardAxis=+Z  TranslationStandardOffset=0  TranslationCartesianOffset=smiData.RigidTransform(511).translation  TranslationROffset=0  TranslationROffsetUnits=m  TranslationZOffset=0  TranslationZOffsetUnits=m  TranslationThetaOffset=0  TranslationThetaOffsetUnits=deg  RotationMethod=ArbitraryAxis  RotationAngleUnits=rad  RotationStandardAxis=+Z  RotationAngle=smiData.RigidTransform(511).angle  RotationArbitraryAxis=smiData.RigidTransform(511).axis  FollAlignAxisA=+X  BaseAlignAxisA=+Y  FollAlignAxisB=+Y  BaseAlignAxisB=+Z  RotationSequenceAxes=FollowerAxes  RotationSequence=XYX  RotationSequenceAngles=[0 0 0]  RotationSequenceAnglesUnits=deg  RotationMatrix=[1 0 0; 0 1 0; 0 0 1]
  Transform85 : sm_lib/Frames and Transforms/Rigid Transform  TranslationMethod=Cartesian  TranslationLengthUnit=in  TranslationStandardAxis=+Z  TranslationStandardOffset=0  TranslationCartesianOffset=smiData.RigidTransform(512).translation  TranslationROffset=0  TranslationROffsetUnits=m  TranslationZOffset=0  TranslationZOffsetUnits=m  TranslationThetaOffset=0  TranslationThetaOffsetUnits=deg  RotationMethod=ArbitraryAxis  RotationAngleUnits=rad  RotationStandardAxis=+Z  RotationAngle=smiData.RigidTransform(512).angle  RotationArbitraryAxis=smiData.RigidTransform(512).axis  FollAlignAxisA=+X  BaseAlignAxisA=+Y  FollAlignAxisB=+Y  BaseAlignAxisB=+Z  RotationSequenceAxes=FollowerAxes  RotationSequence=XYX  RotationSequenceAngles=[0 0 0]  RotationSequenceAnglesUnits=deg  RotationMatrix=[1 0 0; 0 1 0; 0 0 1]
  Transform86 : sm_lib/Frames and Transforms/Rigid Transform  TranslationMethod=Cartesian  TranslationLengthUnit=in  TranslationStandardAxis=+Z  TranslationStandardOffset=0  TranslationCartesianOffset=smiData.RigidTransform(513).translation  TranslationROffset=0  TranslationROffsetUnits=m  TranslationZOffset=0  TranslationZOffsetUnits=m  TranslationThetaOffset=0  TranslationThetaOffsetUnits=deg  RotationMethod=ArbitraryAxis  RotationAngleUnits=rad  RotationStandardAxis=+Z  RotationAngle=smiData.RigidTransform(513).angle  RotationArbitraryAxis=smiData.RigidTransform(513).axis  FollAlignAxisA=+X  BaseAlignAxisA=+Y  FollAlignAxisB=+Y  BaseAlignAxisB=+Z  RotationSequenceAxes=FollowerAxes  RotationSequence=XYX  RotationSequenceAngles=[0 0 0]  RotationSequenceAnglesUnits=deg  RotationMatrix=[1 0 0; 0 1 0; 0 0 1]
  Transform87 : sm_lib/Frames and Transforms/Rigid Transform  TranslationMethod=Cartesian  TranslationLengthUnit=in  TranslationStandardAxis=+Z  TranslationStandardOffset=0  TranslationCartesianOffset=smiData.RigidTransform(514).translation  TranslationROffset=0  TranslationROffsetUnits=m  TranslationZOffset=0  TranslationZOffsetUnits=m  TranslationThetaOffset=0  TranslationThetaOffsetUnits=deg  RotationMethod=ArbitraryAxis  RotationAngleUnits=rad  RotationStandardAxis=+Z  RotationAngle=smiData.RigidTransform(514).angle  RotationArbitraryAxis=smiData.RigidTransform(514).axis  FollAlignAxisA=+X  BaseAlignAxisA=+Y  FollAlignAxisB=+Y  BaseAlignAxisB=+Z  RotationSequenceAxes=FollowerAxes  RotationSequence=XYX  RotationSequenceAngles=[0 0 0]  RotationSequenceAnglesUnits=deg  RotationMatrix=[1 0 0; 0 1 0; 0 0 1]
  Transform88 : sm_lib/Frames and Transforms/Rigid Transform  TranslationMethod=Cartesian  TranslationLengthUnit=in  TranslationStandardAxis=+Z  TranslationStandardOffset=0  TranslationCartesianOffset=smiData.RigidTransform(515).translation  TranslationROffset=0  TranslationROffsetUnits=m  TranslationZOffset=0  TranslationZOffsetUnits=m  TranslationThetaOffset=0  TranslationThetaOffsetUnits=deg  RotationMethod=ArbitraryAxis  RotationAngleUnits=rad  RotationStandardAxis=+Z  RotationAngle=smiData.RigidTransform(515).angle  RotationArbitraryAxis=smiData.RigidTransform(515).axis  FollAlignAxisA=+X  BaseAlignAxisA=+Y  FollAlignAxisB=+Y  BaseAlignAxisB=+Z  RotationSequenceAxes=FollowerAxes  RotationSequence=XYX  RotationSequenceAngles=[0 0 0]  RotationSequenceAnglesUnits=deg  RotationMatrix=[1 0 0; 0 1 0; 0 0 1]
  Transform89 : sm_lib/Frames and Transforms/Rigid Transform  TranslationMethod=Cartesian  TranslationLengthUnit=in  TranslationStandardAxis=+Z  TranslationStandardOffset=0  TranslationCartesianOffset=smiData.RigidTransform(516).translation  TranslationROffset=0  TranslationROffsetUnits=m  TranslationZOffset=0  TranslationZOffsetUnits=m  TranslationThetaOffset=0  TranslationThetaOffsetUnits=deg  RotationMethod=ArbitraryAxis  RotationAngleUnits=rad  RotationStandardAxis=+Z  RotationAngle=smiData.RigidTransform(516).angle  RotationArbitraryAxis=smiData.RigidTransform(516).axis  FollAlignAxisA=+X  BaseAlignAxisA=+Y  FollAlignAxisB=+Y  BaseAlignAxisB=+Z  RotationSequenceAxes=FollowerAxes  RotationSequence=XYX  RotationSequenceAngles=[0 0 0]  RotationSequenceAnglesUnits=deg  RotationMatrix=[1 0 0; 0 1 0; 0 0 1]
  Transform9 : sm_lib/Frames and Transforms/Rigid Transform  TranslationMethod=Cartesian  TranslationLengthUnit=in  TranslationStandardAxis=+Z  TranslationStandardOffset=0  TranslationCartesianOffset=smiData.RigidTransform(436).translation  TranslationROffset=0  TranslationROffsetUnits=m  TranslationZOffset=0  TranslationZOffsetUnits=m  TranslationThetaOffset=0  TranslationThetaOffsetUnits=deg  RotationMethod=ArbitraryAxis  RotationAngleUnits=rad  RotationStandardAxis=+Z  RotationAngle=smiData.RigidTransform(436).angle  RotationArbitraryAxis=smiData.RigidTransform(436).axis  FollAlignAxisA=+X  BaseAlignAxisA=+Y  FollAlignAxisB=+Y  BaseAlignAxisB=+Z  RotationSequenceAxes=FollowerAxes  RotationSequence=XYX  RotationSequenceAngles=[0 0 0]  RotationSequenceAnglesUnits=deg  RotationMatrix=[1 0 0; 0 1 0; 0 0 1]
  Transform90 : sm_lib/Frames and Transforms/Rigid Transform  TranslationMethod=Cartesian  TranslationLengthUnit=in  TranslationStandardAxis=+Z  TranslationStandardOffset=0  TranslationCartesianOffset=smiData.RigidTransform(517).translation  TranslationROffset=0  TranslationROffsetUnits=m  TranslationZOffset=0  TranslationZOffsetUnits=m  TranslationThetaOffset=0  TranslationThetaOffsetUnits=deg  RotationMethod=ArbitraryAxis  RotationAngleUnits=rad  RotationStandardAxis=+Z  RotationAngle=smiData.RigidTransform(517).angle  RotationArbitraryAxis=smiData.RigidTransform(517).axis  FollAlignAxisA=+X  BaseAlignAxisA=+Y  FollAlignAxisB=+Y  BaseAlignAxisB=+Z  RotationSequenceAxes=FollowerAxes  RotationSequence=XYX  RotationSequenceAngles=[0 0 0]  RotationSequenceAnglesUnits=deg  RotationMatrix=[1 0 0; 0 1 0; 0 0 1]
  Transform91 : sm_lib/Frames and Transforms/Rigid Transform  TranslationMethod=Cartesian  TranslationLengthUnit=in  TranslationStandardAxis=+Z  TranslationStandardOffset=0  TranslationCartesianOffset=smiData.RigidTransform(518).translation  TranslationROffset=0  TranslationROffsetUnits=m  TranslationZOffset=0  TranslationZOffsetUnits=m  TranslationThetaOffset=0  TranslationThetaOffsetUnits=deg  RotationMethod=ArbitraryAxis  RotationAngleUnits=rad  RotationStandardAxis=+Z  RotationAngle=smiData.RigidTransform(518).angle  RotationArbitraryAxis=smiData.RigidTransform(518).axis  FollAlignAxisA=+X  BaseAlignAxisA=+Y  FollAlignAxisB=+Y  BaseAlignAxisB=+Z  RotationSequenceAxes=FollowerAxes  RotationSequence=XYX  RotationSequenceAngles=[0 0 0]  RotationSequenceAnglesUnits=deg  RotationMatrix=[1 0 0; 0 1 0; 0 0 1]
  Transform92 : sm_lib/Frames and Transforms/Rigid Transform  TranslationMethod=Cartesian  TranslationLengthUnit=in  TranslationStandardAxis=+Z  TranslationStandardOffset=0  TranslationCartesianOffset=smiData.RigidTransform(519).translation  TranslationROffset=0  TranslationROffsetUnits=m  TranslationZOffset=0  TranslationZOffsetUnits=m  TranslationThetaOffset=0  TranslationThetaOffsetUnits=deg  RotationMethod=ArbitraryAxis  RotationAngleUnits=rad  RotationStandardAxis=+Z  RotationAngle=smiData.RigidTransform(519).angle  RotationArbitraryAxis=smiData.RigidTransform(519).axis  FollAlignAxisA=+X  BaseAlignAxisA=+Y  FollAlignAxisB=+Y  BaseAlignAxisB=+Z  RotationSequenceAxes=FollowerAxes  RotationSequence=XYX  RotationSequenceAngles=[0 0 0]  RotationSequenceAnglesUnits=deg  RotationMatrix=[1 0 0; 0 1 0; 0 0 1]
  Transform93 : sm_lib/Frames and Transforms/Rigid Transform  TranslationMethod=Cartesian  TranslationLengthUnit=in  TranslationStandardAxis=+Z  TranslationStandardOffset=0  TranslationCartesianOffset=smiData.RigidTransform(520).translation  TranslationROffset=0  TranslationROffsetUnits=m  TranslationZOffset=0  TranslationZOffsetUnits=m  TranslationThetaOffset=0  TranslationThetaOffsetUnits=deg  RotationMethod=ArbitraryAxis  RotationAngleUnits=rad  RotationStandardAxis=+Z  RotationAngle=smiData.RigidTransform(520).angle  RotationArbitraryAxis=smiData.RigidTransform(520).axis  FollAlignAxisA=+X  BaseAlignAxisA=+Y  FollAlignAxisB=+Y  BaseAlignAxisB=+Z  RotationSequenceAxes=FollowerAxes  RotationSequence=XYX  RotationSequenceAngles=[0 0 0]  RotationSequenceAnglesUnits=deg  RotationMatrix=[1 0 0; 0 1 0; 0 0 1]
  Transform94 : sm_lib/Frames and Transforms/Rigid Transform  TranslationMethod=Cartesian  TranslationLengthUnit=in  TranslationStandardAxis=+Z  TranslationStandardOffset=0  TranslationCartesianOffset=smiData.RigidTransform(521).translation  TranslationROffset=0  TranslationROffsetUnits=m  TranslationZOffset=0  TranslationZOffsetUnits=m  TranslationThetaOffset=0  TranslationThetaOffsetUnits=deg  RotationMethod=ArbitraryAxis  RotationAngleUnits=rad  RotationStandardAxis=+Z  RotationAngle=smiData.RigidTransform(521).angle  RotationArbitraryAxis=smiData.RigidTransform(521).axis  FollAlignAxisA=+X  BaseAlignAxisA=+Y  FollAlignAxisB=+Y  BaseAlignAxisB=+Z  RotationSequenceAxes=FollowerAxes  RotationSequence=XYX  RotationSequenceAngles=[0 0 0]  RotationSequenceAnglesUnits=deg  RotationMatrix=[1 0 0; 0 1 0; 0 0 1]
  Transform95 : sm_lib/Frames and Transforms/Rigid Transform  TranslationMethod=Cartesian  TranslationLengthUnit=in  TranslationStandardAxis=+Z  TranslationStandardOffset=0  TranslationCartesianOffset=smiData.RigidTransform(522).translation  TranslationROffset=0  TranslationROffsetUnits=m  TranslationZOffset=0  TranslationZOffsetUnits=m  TranslationThetaOffset=0  TranslationThetaOffsetUnits=deg  RotationMethod=ArbitraryAxis  RotationAngleUnits=rad  RotationStandardAxis=+Z  RotationAngle=smiData.RigidTransform(522).angle  RotationArbitraryAxis=smiData.RigidTransform(522).axis  FollAlignAxisA=+X  BaseAlignAxisA=+Y  FollAlignAxisB=+Y  BaseAlignAxisB=+Z  RotationSequenceAxes=FollowerAxes  RotationSequence=XYX  RotationSequenceAngles=[0 0 0]  RotationSequenceAnglesUnits=deg  RotationMatrix=[1 0 0; 0 1 0; 0 0 1]
  Transform96 : sm_lib/Frames and Transforms/Rigid Transform  TranslationMethod=Cartesian  TranslationLengthUnit=in  TranslationStandardAxis=+Z  TranslationStandardOffset=0  TranslationCartesianOffset=smiData.RigidTransform(523).translation  TranslationROffset=0  TranslationROffsetUnits=m  TranslationZOffset=0  TranslationZOffsetUnits=m  TranslationThetaOffset=0  TranslationThetaOffsetUnits=deg  RotationMethod=ArbitraryAxis  RotationAngleUnits=rad  RotationStandardAxis=+Z  RotationAngle=smiData.RigidTransform(523).angle  RotationArbitraryAxis=smiData.RigidTransform(523).axis  FollAlignAxisA=+X  BaseAlignAxisA=+Y  FollAlignAxisB=+Y  BaseAlignAxisB=+Z  RotationSequenceAxes=FollowerAxes  RotationSequence=XYX  RotationSequenceAngles=[0 0 0]  RotationSequenceAnglesUnits=deg  RotationMatrix=[1 0 0; 0 1 0; 0 0 1]
  Transform97 : sm_lib/Frames and Transforms/Rigid Transform  TranslationMethod=Cartesian  TranslationLengthUnit=in  TranslationStandardAxis=+Z  TranslationStandardOffset=0  TranslationCartesianOffset=smiData.RigidTransform(524).translation  TranslationROffset=0  TranslationROffsetUnits=m  TranslationZOffset=0  TranslationZOffsetUnits=m  TranslationThetaOffset=0  TranslationThetaOffsetUnits=deg  RotationMethod=ArbitraryAxis  RotationAngleUnits=rad  RotationStandardAxis=+Z  RotationAngle=smiData.RigidTransform(524).angle  RotationArbitraryAxis=smiData.RigidTransform(524).axis  FollAlignAxisA=+X  BaseAlignAxisA=+Y  FollAlignAxisB=+Y  BaseAlignAxisB=+Z  RotationSequenceAxes=FollowerAxes  RotationSequence=XYX  RotationSequenceAngles=[0 0 0]  RotationSequenceAnglesUnits=deg  RotationMatrix=[1 0 0; 0 1 0; 0 0 1]
  Transform98 : sm_lib/Frames and Transforms/Rigid Transform  TranslationMethod=Cartesian  TranslationLengthUnit=in  TranslationStandardAxis=+Z  TranslationStandardOffset=0  TranslationCartesianOffset=smiData.RigidTransform(525).translation  TranslationROffset=0  TranslationROffsetUnits=m  TranslationZOffset=0  TranslationZOffsetUnits=m  TranslationThetaOffset=0  TranslationThetaOffsetUnits=deg  RotationMethod=ArbitraryAxis  RotationAngleUnits=rad  RotationStandardAxis=+Z  RotationAngle=smiData.RigidTransform(525).angle  RotationArbitraryAxis=smiData.RigidTransform(525).axis  FollAlignAxisA=+X  BaseAlignAxisA=+Y  FollAlignAxisB=+Y  BaseAlignAxisB=+Z  RotationSequenceAxes=FollowerAxes  RotationSequence=XYX  RotationSequenceAngles=[0 0 0]  RotationSequenceAnglesUnits=deg  RotationMatrix=[1 0 0; 0 1 0; 0 0 1]
  Transform99 : sm_lib/Frames and Transforms/Rigid Transform  TranslationMethod=Cartesian  TranslationLengthUnit=in  TranslationStandardAxis=+Z  TranslationStandardOffset=0  TranslationCartesianOffset=smiData.RigidTransform(526).translation  TranslationROffset=0  TranslationROffsetUnits=m  TranslationZOffset=0  TranslationZOffsetUnits=m  TranslationThetaOffset=0  TranslationThetaOffsetUnits=deg  RotationMethod=ArbitraryAxis  RotationAngleUnits=rad  RotationStandardAxis=+Z  RotationAngle=smiData.RigidTransform(526).angle  RotationArbitraryAxis=smiData.RigidTransform(526).axis  FollAlignAxisA=+X  BaseAlignAxisA=+Y  FollAlignAxisB=+Y  BaseAlignAxisB=+Z  RotationSequenceAxes=FollowerAxes  RotationSequence=XYX  RotationSequenceAngles=[0 0 0]  RotationSequenceAnglesUnits=deg  RotationMatrix=[1 0 0; 0 1 0; 0 0 1]
  VFQFPN48_OPL6206QTR_1_RIGID : Subsystem
  VSSOP8_LOGICNOTSN74LVC3G14DCU_1_RIGID : Subsystem
  VSSOP8_LOGICNOTSN74LVC3G14DCU_2_RIGID : Subsystem
  x0402CAP_COMMON_10_RIGID : Subsystem
  x0402CAP_COMMON_11_RIGID : Subsystem
  x0402CAP_COMMON_12_RIGID : Subsystem
  x0402CAP_COMMON_13_RIGID : Subsystem
  x0402CAP_COMMON_14_RIGID : Subsystem
  x0402CAP_COMMON_15_RIGID : Subsystem
  x0402CAP_COMMON_16_RIGID : Subsystem
  x0402CAP_COMMON_17_RIGID : Subsystem
  x0402CAP_COMMON_18_RIGID : Subsystem
  x0402CAP_COMMON_19_RIGID : Subsystem
  x0402CAP_COMMON_1_RIGID : Subsystem
  x0402CAP_COMMON_20_RIGID : Subsystem
  x0402CAP_COMMON_21_RIGID : Subsystem
  x0402CAP_COMMON_22_RIGID : Subsystem
  x0402CAP_COMMON_23_RIGID : Subsystem
  x0402CAP_COMMON_24_RIGID : Subsystem
  x0402CAP_COMMON_25_RIGID : Subsystem
  x0402CAP_COMMON_26_RIGID : Subsystem
  x0402CAP_COMMON_27_RIGID : Subsystem
  x0402CAP_COMMON_28_RIGID : Subsystem
  x0402CAP_COMMON_29_RIGID : Subsystem
  x0402CAP_COMMON_2_RIGID : Subsystem
  x0402CAP_COMMON_30_RIGID : Subsystem
  x0402CAP_COMMON_31_RIGID : Subsystem
  x0402CAP_COMMON_32_RIGID : Subsystem
  x0402CAP_COMMON_33_RIGID : Subsystem
  x0402CAP_COMMON_34_RIGID : Subsystem
  x0402CAP_COMMON_35_RIGID : Subsystem
  x0402CAP_COMMON_36_RIGID : Subsystem
  x0402CAP_COMMON_37_RIGID : Subsystem
  x0402CAP_COMMON_38_RIGID : Subsystem
  x0402CAP_COMMON_39_RIGID : Subsystem
  x0402CAP_COMMON_3_RIGID : Subsystem
  x0402CAP_COMMON_40_RIGID : Subsystem
  x0402CAP_COMMON_4_RIGID : Subsystem
  x0402CAP_COMMON_5_RIGID : Subsystem
  x0402CAP_COMMON_6_RIGID : Subsystem
  x0402CAP_COMMON_7_RIGID : Subsystem
  x0402CAP_COMMON_8_RIGID : Subsystem
  x0402CAP_COMMON_9_RIGID : Subsystem
  x0402RES_COMMON_10_RIGID : Subsystem
  x0402RES_COMMON_11_RIGID : Subsystem
  x0402RES_COMMON_12_RIGID : Subsystem
  x0402RES_COMMON_13_RIGID : Subsystem
  x0402RES_COMMON_14_RIGID : Subsystem
  x0402RES_COMMON_15_RIGID : Subsystem
  x0402RES_COMMON_16_RIGID : Subsystem
  x0402RES_COMMON_17_RIGID : Subsystem
  x0402RES_COMMON_1_RIGID : Subsystem
  x0402RES_COMMON_2_RIGID : Subsystem
  x0402RES_COMMON_3_RIGID : Subsystem
  x0402RES_COMMON_4_RIGID : Subsystem
  x0402RES_COMMON_5_RIGID : Subsystem
  x0402RES_COMMON_6_RIGID : Subsystem
  x0402RES_COMMON_7_RIGID : Subsystem
  x0402RES_COMMON_8_RIGID : Subsystem
  x0402RES_COMMON_9_RIGID : Subsystem
  x0603CAP_COMMON_1_RIGID : Subsystem
  x0603CAP_COMMON_2_RIGID : Subsystem
  x0603CAP_COMMON_3_RIGID : Subsystem
  x0603CAP_COMMON_4_RIGID : Subsystem
  x0603CAP_COMMON_5_RIGID : Subsystem
  x0603CAP_COMMON_6_RIGID : Subsystem
  x0603CAP_COMMON_7_RIGID : Subsystem
  x0603CAP_COMMON_8_RIGID : Subsystem
  x0603RES_COMMON_1_RIGID : Subsystem
  x2512RES_COMMON_1_RIGID : Subsystem
  x2512RES_COMMON_2_RIGID : Subsystem
  x2512RES_COMMON_3_RIGID : Subsystem
  x2512RES_COMMON_4_RIGID : Subsystem
  x2512RES_COMMON_5_RIGID : Subsystem
  F : PMIOPort  Port=1  Side=Right
  connections:
  Transform/RConn1 -- x0402CAP_COMMON_37_RIGID/LConn1
  Transform1/RConn1 -- x0402CAP_COMMON_20_RIGID/LConn1
  Transform10/RConn1 -- x0402CAP_COMMON_14_RIGID/LConn1
  Transform100/RConn1 -- x2512RES_COMMON_1_RIGID/LConn1
  Transform101/RConn1 -- x2512RES_COMMON_2_RIGID/LConn1
  Transform102/RConn1 -- x2512RES_COMMON_3_RIGID/LConn1
  Transform103/RConn1 -- x2512RES_COMMON_4_RIGID/LConn1
  Transform104/RConn1 -- x2512RES_COMMON_5_RIGID/LConn1
  MSOP10_COMMON_1_RIGID/LConn1 -- Transform105/RConn1
  Transform/LConn1 -- ReferenceFrame/RConn1 -- Transform1/LConn1 -- Transform10/LConn1 -- Transform100/LConn1 -- Transform101/LConn1 -- Transform102/LConn1 -- Transform103/LConn1 -- Transform104/LConn1 -- Transform105/LConn1 -- Transform106/RConn1 -- Transform11/LConn1 -- Transform12/LConn1 -- Transform13/LConn1 -- Transform14/LConn1 -- Transform15/LConn1 -- Transform16/LConn1 -- Transform17/LConn1 -- Transform18/LConn1 -- Transform19/LConn1 -- Transform2/LConn1 -- Transform20/LConn1 -- Transform21/LConn1 -- Transform22/LConn1 -- Transform23/LConn1 -- Transform24/LConn1 -- Transform25/LConn1 -- Transform26/LConn1 -- Transform27/LConn1 -- Transform28/LConn1 -- Transform29/LConn1 -- Transform3/LConn1 -- Transform30/LConn1 -- Transform31/LConn1 -- Transform32/LConn1 -- Transform33/LConn1 -- Transform34/LConn1 -- Transform35/LConn1 -- Transform36/LConn1 -- Transform37/LConn1 -- Transform38/LConn1 -- Transform39/LConn1 -- Transform4/LConn1 -- Transform40/LConn1 -- Transform41/LConn1 -- Transform42/LConn1 -- Transform43/LConn1 -- Transform44/LConn1 -- Transform45/LConn1 -- Transform46/LConn1 -- Transform47/LConn1 -- Transform48/LConn1 -- Transform49/LConn1 -- Transform5/LConn1 -- Transform50/LConn1 -- Transform51/LConn1 -- Transform52/LConn1 -- Transform53/LConn1 -- Transform54/LConn1 -- Transform55/LConn1 -- Transform56/LConn1 -- Transform57/LConn1 -- Transform58/LConn1 -- Transform59/LConn1 -- Transform6/LConn1 -- Transform60/LConn1 -- Transform61/LConn1 -- Transform62/LConn1 -- Transform63/LConn1 -- Transform64/LConn1 -- Transform65/LConn1 -- Transform66/LConn1 -- Transform67/LConn1 -- Transform68/LConn1 -- Transform69/LConn1 -- Transform7/LConn1 -- Transform70/LConn1 -- Transform71/LConn1 -- Transform72/LConn1 -- Transform73/LConn1 -- Transform74/LConn1 -- Transform75/LConn1 -- Transform76/LConn1 -- Transform77/LConn1 -- Transform78/LConn1 -- Transform79/LConn1 -- Transform8/LConn1 -- Transform80/LConn1 -- Transform81/LConn1 -- Transform82/LConn1 -- Transform83/LConn1 -- Transform84/LConn1 -- Transform85/LConn1 -- Transform86/LConn1 -- Transform87/LConn1 -- Transform88/LConn1 -- Transform89/LConn1 -- Transform9/LConn1 -- Transform90/LConn1 -- Transform91/LConn1 -- Transform92/LConn1 -- Transform93/LConn1 -- Transform94/LConn1 -- Transform95/LConn1 -- Transform96/LConn1 -- Transform97/LConn1 -- Transform98/LConn1 -- Transform99/LConn1
  Transform106/LConn1 -- F/RConn1
  Transform11/RConn1 -- x0402CAP_COMMON_12_RIGID/LConn1
  Transform12/RConn1 -- x0402CAP_COMMON_16_RIGID/LConn1
  Transform13/RConn1 -- x0402CAP_COMMON_15_RIGID/LConn1
  Transform14/RConn1 -- x0402CAP_COMMON_18_RIGID/LConn1
  Transform15/RConn1 -- x0402CAP_COMMON_27_RIGID/LConn1
  Transform16/RConn1 -- x0402CAP_COMMON_29_RIGID/LConn1
  Transform17/RConn1 -- x0402CAP_COMMON_28_RIGID/LConn1
  Transform18/RConn1 -- x0402CAP_COMMON_26_RIGID/LConn1
  Transform19/RConn1 -- x0402CAP_COMMON_25_RIGID/LConn1
  Transform2/RConn1 -- x0402CAP_COMMON_21_RIGID/LConn1
  Transform20/RConn1 -- x0402CAP_COMMON_7_RIGID/LConn1
  Transform21/RConn1 -- x0402RES_COMMON_14_RIGID/LConn1
  Transform22/RConn1 -- x0402RES_COMMON_17_RIGID/LConn1
  Transform23/RConn1 -- x0402RES_COMMON_4_RIGID/LConn1
  Transform24/RConn1 -- x0402RES_COMMON_2_RIGID/LConn1
  Transform25/RConn1 -- x0402RES_COMMON_16_RIGID/LConn1
  Transform26/RConn1 -- x0402CAP_COMMON_9_RIGID/LConn1
  Transform27/RConn1 -- x0402RES_COMMON_13_RIGID/LConn1
  Transform28/RConn1 -- x0402RES_COMMON_12_RIGID/LConn1
  Transform29/RConn1 -- x0402RES_COMMON_8_RIGID/LConn1
  Transform3/RConn1 -- x0402CAP_COMMON_23_RIGID/LConn1
  Transform30/RConn1 -- x0402RES_COMMON_15_RIGID/LConn1
  Transform31/RConn1 -- x0402RES_COMMON_5_RIGID/LConn1
  Transform32/RConn1 -- x0402RES_COMMON_6_RIGID/LConn1
  Transform33/RConn1 -- x0402CAP_COMMON_2_RIGID/LConn1
  Transform34/RConn1 -- x0402CAP_COMMON_6_RIGID/LConn1
  Transform35/RConn1 -- x0402RES_COMMON_10_RIGID/LConn1
  Transform36/RConn1 -- x0402CAP_COMMON_10_RIGID/LConn1
  Transform37/RConn1 -- x0402RES_COMMON_3_RIGID/LConn1
  Transform38/RConn1 -- x0402RES_COMMON_9_RIGID/LConn1
  Transform39/RConn1 -- x0402CAP_COMMON_4_RIGID/LConn1
  Transform4/RConn1 -- x0402CAP_COMMON_22_RIGID/LConn1
  Transform40/RConn1 -- x0402RES_COMMON_11_RIGID/LConn1
  Transform41/RConn1 -- x0402CAP_COMMON_3_RIGID/LConn1
  Transform42/RConn1 -- x0402RES_COMMON_7_RIGID/LConn1
  Transform43/RConn1 -- x0402CAP_COMMON_5_RIGID/LConn1
  Transform44/RConn1 -- x0402CAP_COMMON_8_RIGID/LConn1
  Transform45/RConn1 -- x0402CAP_COMMON_1_RIGID/LConn1
  Transform46/RConn1 -- x0402CAP_COMMON_31_RIGID/LConn1
  Transform47/RConn1 -- x0402CAP_COMMON_32_RIGID/LConn1
  Transform48/RConn1 -- x0402CAP_COMMON_33_RIGID/LConn1
  Transform49/RConn1 -- x0402CAP_COMMON_34_RIGID/LConn1
  Transform5/RConn1 -- x0402CAP_COMMON_24_RIGID/LConn1
  Transform50/RConn1 -- x0402CAP_COMMON_30_RIGID/LConn1
  Transform51/RConn1 -- x0402CAP_COMMON_36_RIGID/LConn1
  Transform52/RConn1 -- x0402CAP_COMMON_35_RIGID/LConn1
  CONNMDF3A9P2DS_CONNMDF3A9P2DS_1_RIGID/LConn1 -- Transform53/RConn1
  RARRAYYC124_RA40R0_3_RIGID/LConn1 -- Transform54/RConn1
  TP16258543_TP16258543_6_RIGID/LConn1 -- Transform55/RConn1
  SOT235_COMMON_1_RIGID/LConn1 -- Transform56/RConn1
  Transform57/RConn1 -- VSSOP8_LOGICNOTSN74LVC3G14DCU_2_RIGID/LConn1
  RARRAYYC124_RA41K005_2_RIGID/LConn1 -- Transform58/RConn1
  MSOP8Q_AICAD8418WBRMZ_2_RIGID/LConn1 -- Transform59/RConn1
  Transform6/RConn1 -- x0402CAP_COMMON_13_RIGID/LConn1
  SOT235_COMMON_2_RIGID/LConn1 -- Transform60/RConn1
  TP16258543_TP16258543_2_RIGID/LConn1 -- Transform61/RConn1
  Transform62/RConn1 -- x0402RES_COMMON_1_RIGID/LConn1
  RARRAYYC124_RA41K005_1_RIGID/LConn1 -- Transform63/RConn1
  CONNMDF3A6P2DS_CONNMDF3A6P2DS_1_RIGID/LConn1 -- Transform64/RConn1
  CEEEFC1H101P_C100U50VEEEFC1H101P_1_RIGID/LConn1 -- Transform65/RConn1
  C006_285_1_RIGID/LConn1 -- Transform66/RConn1
  TP16258543_TP16258543_1_RIGID/LConn1 -- Transform67/RConn1
  TP16258543_TP16258543_3_RIGID/LConn1 -- Transform68/RConn1
  RARRAYYC124_RA40R0_2_RIGID/LConn1 -- Transform69/RConn1
  Transform7/RConn1 -- x0402CAP_COMMON_17_RIGID/LConn1
  TP16258543_TP16258543_5_RIGID/LConn1 -- Transform70/RConn1
  TP16258543_TP16258543_4_RIGID/LConn1 -- Transform71/RConn1
  OSCECS20xx_OSC40000MHZ_1_RIGID/LConn1 -- Transform72/RConn1
  Transform73/RConn1 -- VFQFPN48_OPL6206QTR_1_RIGID/LConn1
  RARRAYYC124_RA40R0_1_RIGID/LConn1 -- Transform74/RConn1
  Transform75/RConn1 -- VSSOP8_LOGICNOTSN74LVC3G14DCU_1_RIGID/LConn1
  MSOP8Q_AICAD8418WBRMZ_1_RIGID/LConn1 -- Transform76/RConn1
  TQFP144Max_V_CPLD_ground_pins_CPLD5M1270ZT144C5N_1_RIGID/LConn1 -- Transform77/RConn1
  RARRAYYC124_RA40R0_4_RIGID/LConn1 -- Transform78/RConn1
  MSOP8Q_AICAD8418WBRMZ_3_RIGID/LConn1 -- Transform79/RConn1
  Transform8/RConn1 -- x0402CAP_COMMON_11_RIGID/LConn1
  MSOP8Q_AICAD8418WBRMZ_4_RIGID/LConn1 -- Transform80/RConn1
  CONNMDF3A6P2DS_CONNMDF3A6P2DS_2_RIGID/LConn1 -- Transform81/RConn1
  DDO214AB_DB560C13F_1_RIGID/LConn1 -- Transform82/RConn1
  LGA16_3x3x086mm_ACCGYROLSM6DS0_1_RIGID/LConn1 -- Transform83/RConn1
  DDO214AA_DSMBJ5361BTP_1_RIGID/LConn1 -- Transform84/RConn1
  Transform85/RConn1 -- x0402CAP_COMMON_38_RIGID/LConn1
  Transform86/RConn1 -- x0402CAP_COMMON_39_RIGID/LConn1
  Transform87/RConn1 -- x0402CAP_COMMON_40_RIGID/LConn1
  Transform88/RConn1 -- x0603RES_COMMON_1_RIGID/LConn1
  Transform89/RConn1 -- x0603CAP_COMMON_1_RIGID/LConn1
  Transform9/RConn1 -- x0402CAP_COMMON_19_RIGID/LConn1
  Transform90/RConn1 -- x0603CAP_COMMON_2_RIGID/LConn1
  Transform91/RConn1 -- x0603CAP_COMMON_3_RIGID/LConn1
  Transform92/RConn1 -- x0603CAP_COMMON_4_RIGID/LConn1
  Transform93/RConn1 -- x0603CAP_COMMON_5_RIGID/LConn1
  Transform94/RConn1 -- x0603CAP_COMMON_6_RIGID/LConn1
  Transform95/RConn1 -- x0603CAP_COMMON_7_RIGID/LConn1
  Transform96/RConn1 -- x0603CAP_COMMON_8_RIGID/LConn1
  SOT23_COMMON_1_RIGID/LConn1 -- Transform97/RConn1
  SOT23_COMMON_2_RIGID/LConn1 -- Transform98/RConn1
  SOT23_COMMON_3_RIGID/LConn1 -- Transform99/RConn1
